simulink model "EV_Modeling"  (R2024b)
settings: Solver=FixedStepAuto  StartTime=0.0  StopTime=3500  FixedStep=0.1  RelTol=1e-3
values from neighbouring files (symbols this model uses):
  battery_SOC_resistance = battery_SOC(:,3)    [EV_Truck.m]
  battery_SOC_SOC = battery_SOC(:,1)    [EV_Truck.m]    (also in simulink.m)
  battery_SOC_voltage = battery_SOC(:,2)    [EV_Truck.m]    (also in simulink.m)
  electric_consumption_ressistancce = electric_consumption(:,2)    [EV_Truck.m]    (also in simulink.m)
  electric_consumption_voltage = electric_consumption(:,1)    [EV_Truck.m]    (also in simulink.m)
  motor_efficiency_efficiency = table2array(motor_efficiency(2:height(motor_efficiency),2:width(motor_efficiency)))    [EV_Truck.m]    (also in simulink.m)
  motor_efficiency_RPM = table2array(motor_efficiency(2:height(motor_efficiency),1))    [EV_Truck.m]    (also in simulink.m)
  motor_efficiency_torque = transpose(motor_efficiency_torque)    [EV_Truck.m]    (also in simulink.m)
  motor_RPM_torque = table2array(motor_torque(1:14,1))    [EV_Truck.m]    (also in simulink.m)
  motor_torque_RPM = table2array(motor_torque(1:14,2))    [EV_Truck.m]    (also in simulink.m)
undefined symbols (not defined in the file or in its folder): battery_builder_rtmsupport, battery_sli_rtmsupport, DiscIntNeverNeededParam, gcbh, recurrentNet
libraries: dlutilitylib x10, dlsequencelib x10, packLibrary_lib x10, simulink x7, dlconvfclib x6, dlactivationlib x5, sharedTrackingLibrary x3, mpcadaslib x2, nesl_utility x2, fl_lib x2, slpidlib x2, simulink_extras x1
(part 6 of 9)

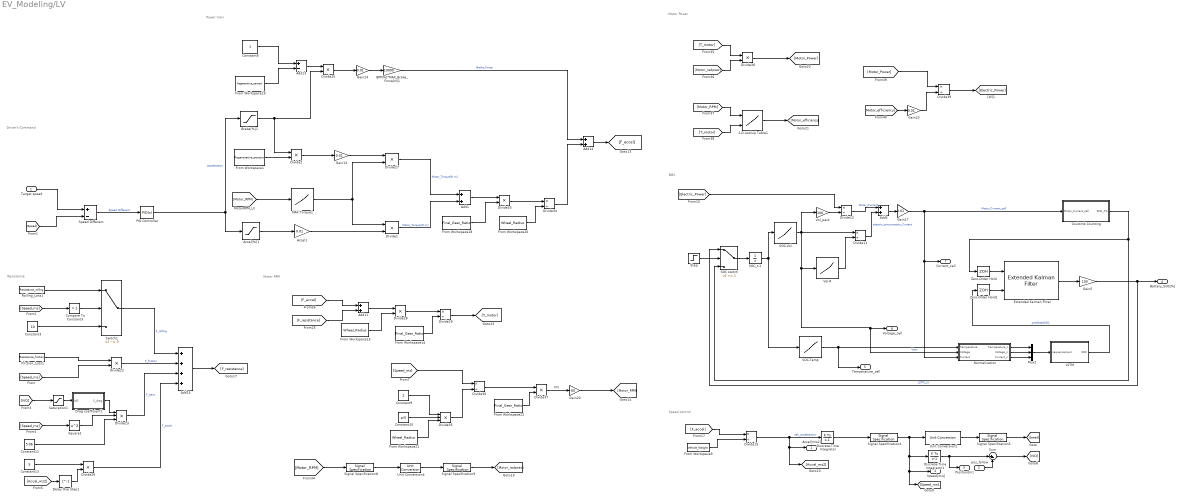
== system EV_Modeling/LV ==
  note: Speed control
  note: Driver's Command
  note: BMS
  note: RPS
  note: Power train
  note: Resistance
  note: Motor RPM
  note: Motor Power
  Target speed : Inport
  pos_follow : Inport  Port=2
  " Normalization" : MATLAB Function  TreatAsAtomicUnit=on
  2-D Lookup Table1 : Lookup_n-D  BreakpointsForDimension1=motor_efficiency_RPM  BreakpointsForDimension2=motor_efficiency_torque  Table=motor_efficiency_efficiency  RemoveProtectionInput=on  InternalRulePriority=Speed  RndMeth=Simplest
      settings: InputPortMap=u0,u1
  Accel1 : Gain  Gain=0.01
  Accel[%]1 : Saturate  UpperLimit=100  LowerLimit=0
  Add{1,4,11,14} (4 alike) : Sum
  Add13 : Sum  Inputs=+-
  Add15 : Sum  Inputs=++++
  BPP[%]*MAX_Brake_Force[N]1 : Gain  Gain=10000
  Brake[%]1 : Saturate  UpperLimit=0  LowerLimit=-100
  Compare To Constant3 : simulink/Logic and Bit Operations/Compare To Constant  relop=>  const=1  OutDataTypeStr=boolean
  Constant10 : Constant  Value=pi()
  Constant12 : Constant  Value=5.06
  Constant13 : Constant  Value=5
  Constant3 : Constant  Value=10
  Constant8 : Constant
  Constant9 : Constant  Value=2
  Coulomb Counting : Subsystem
  Delay One Step1 : Delay  DelayLength=1
  Discrete-Time Integrator : DiscreteIntegrator  SampleTime=-1  ICPrevOutput=DiscIntNeverNeededParam  ICPrevScaledInput=DiscIntNeverNeededParam
  Discrete-Time Integrator1 : DiscreteIntegrator  SampleTime=-1  ICPrevOutput=DiscIntNeverNeededParam  ICPrevScaledInput=DiscIntNeverNeededParam
  Divide{1..2,22,25..28,33,37..38} (10 alike) : Product  Inputs=**
  Divide{11..12,15,29,34,36,39} (7 alike) : Product  Inputs=*/
  Divide23 : Product  Inputs=***
  Divide35 : Product  Inputs=***
  Drag coefficient1 : MATLAB Function  TreatAsAtomicUnit=on
  Extended Kalman Filter : sharedTrackingLibrary/Extended Kalman Filter  StateTransitionFcn=myStateTransitionFcn  HasStateTransitionJacobianFcn=off  HasAdditiveProcessNoise=Additive  ProcessNoise=0.0005  HasTimeVaryingProcessNoise=off  HasStateTransitionFcnExtraArgument=1  InitialState=1  InitialStateCovariance=0.02  MeasurementFcn1=myMeasurementFcn  HasMeasurementJacobianFcn1=off  HasMeasurementEnablePort1=off  HasAdditiveMeasurementNoise1=Additive  MeasurementNoise1=0.01  HasTimeVaryingMeasurementNoise1=off  HasMeasurementFcnExtraArgument1=0  HasMeasurementWrapping1=off  MeasurementFcn2=myMeasurementFcn  HasMeasurementJacobianFcn2=off  HasMeasurementEnablePort2=off  HasAdditiveMeasurementNoise2=Additive  MeasurementNoise2=1  HasTimeVaryingMeasurementNoise2=off  HasMeasurementFcnExtraArgument2=0  HasMeasurementWrapping2=off  MeasurementFcn3=myMeasurementFcn  HasMeasurementJacobianFcn3=off  HasMeasurementEnablePort3=off  HasAdditiveMeasurementNoise3=Additive  MeasurementNoise3=1  HasTimeVaryingMeasurementNoise3=off  HasMeasurementFcnExtraArgument3=0  HasMeasurementWrapping3=off  MeasurementFcn4=myMeasurementFcn  HasMeasurementJacobianFcn4=off  HasMeasurementEnablePort4=off  HasAdditiveMeasurementNoise4=Additive  MeasurementNoise4=1  HasTimeVaryingMeasurementNoise4=off  HasMeasurementFcnExtraArgument4=0  HasMeasurementWrapping4=off  MeasurementFcn5=myMeasurementFcn  HasMeasurementJacobianFcn5=off  HasMeasurementEnablePort5=off  HasAdditiveMeasurementNoise5=Additive  MeasurementNoise5=1  HasTimeVaryingMeasurementNoise5=off  HasMeasurementFcnExtraArgument5=0  HasMeasurementWrapping5=off  EnableMultirate=off  StateTransitionFcnSampleTime=1  MeasurementFcn1SampleTime=1  MeasurementFcn2SampleTime=1  MeasurementFcn3SampleTime=1  MeasurementFcn4SampleTime=1  MeasurementFcn5SampleTime=1  UseCurrentEstimator=on  OutputStateCovariance=off  DataType=double  SampleTime=0.1  NumberOfMeasurements=1
  Friction_Loss1 : FromWorkspace  VariableName=Resistance_friction
  From Workspace1 : FromWorkspace  VariableName=Regenerative_percent
  From Workspace14 : FromWorkspace  VariableName=Final_Gear_Ratio
  From Workspace15 : FromWorkspace  VariableName=Wheel_Radius
  From Workspace18 : FromWorkspace  VariableName=Final_Gear_Ratio
  From Workspace19 : FromWorkspace  VariableName=Regenerative_percent
  From Workspace20 : FromWorkspace  VariableName=Wheel_Radius
  From Workspace21 : FromWorkspace  VariableName=Wheel_Radius
  From Workspace22 : FromWorkspace  VariableName=Final_Gear_Ratio
  From Workspace9 : FromWorkspace  VariableName=Vehicle_Weight
  Gain{13..14,17,23} (4 alike) : Gain  Gain=0.01
  Gain20 : Gain  Gain=60
  Gain5 : Gain  Gain=100
  LSTM : Subsystem  TreatAsAtomicUnit=on
  MAX Torque1 : Lookup_n-D  NumberOfTableDimensions=1  BreakpointsForDimension1=motor_RPM_torque  Table=motor_torque_RPM  RemoveProtectionInput=on  InternalRulePriority=Speed  RndMeth=Simplest
  Mux2 : Mux  Inputs=3
  PID Controller : slpidlib/PID Controller  Controller=PID  Form=Parallel  TimeDomain=Continuous-time  UseExternalTs=off  SampleTime=-1  IntegratorMethod=Forward Euler  FilterMethod=Forward Euler  ControllerParametersSource=internal  P=100  I=0.01  UseKiTs=off  D=0.0001  UseExternalDerivativeSource=off  N=10  UseFilter=on  TunerSelectOption=Transfer Function Based (PID Tuner App)  InitialConditionSource=internal  InitialConditionForIntegrator=0  InitialConditionForFilter=0  DifferentiatorICPrevScaledInput=0  ExternalReset=none  TrackingMode=off  Kt=1  LimitOutput=off  SatLimitsSource=internal  UpperSaturationLimit=inf  LowerSaturationLimit=-inf  LinearizeAsGain=on  AntiWindupMode=none  Kb=1  LimitIntegrator=off  UpperIntegratorSaturationLimit=inf  LowerIntegratorSaturationLimit=-inf  POutMin=[]  POutMax=[]  IOutMin=[]  IOutMax=[]  DOutMin=[]  DOutMax=[]  NOutMin=[]  NOutMax=[]  SumOutMin=[]  SumOutMax=[]  SaturationOutMin=[]  SaturationOutMax=[]  PParamMin=[]  PParamMax=[]  IParamMin=[]  IParamMax=[]  DParamMin=[]  DParamMax=[]  NParamMin=[]  NParamMax=[]  KbParamMin=[]  KbParamMax=[]  KtParamMin=[]  KtParamMax=[]  KbOutMin=[]  KbOutMax=[]  KtOutMin=[]  KtOutMax=[]  IntegratorOutMin=[]  IntegratorOutMax=[]  FilterOutMin=[]  FilterOutMax=[]  SumI1OutMin=[]  SumI1OutMax=[]  SumI2OutMin=[]  SumI2OutMax=[]  SumI3OutMin=[]  SumI3OutMax=[]  SumI4OutMin=[]  SumI4OutMax=[]  SumDOutMin=[]  SumDOutMax=[]  DifferentiatorOutMin=[]  DifferentiatorOutMax=[]  FilterDiffOutCoefMin=[]  FilterDiffOutCoefMax=[]  ReciprocalOutMin=[]  ReciprocalOutMax=[]  SumDenOutMin=[]  SumDenOutMax=[]  SumNumOutMin=[]  SumNumOutMax=[]  DivideOutMin=[]  DivideOutMax=[]  UdiffTsProdOutMin=[]  UdiffTsProdOutMax=[]  NTsProdOutMin=[]  NTsProdOutMax=[]  UintegralTsProdOutMin=[]  UintegralTsProdOutMax=[]  UngainTsProdOutMin=[]  UngainTsProdOutMax=[]  ClampingZeroOutDataTypeStr=Inherit: Inherit via back propagation  ClampingZeroOutMin=[]  ClampingZeroOutMax=[]  FilterDenConstantOutDataTypeStr=Inherit: Inherit via back propagation  FilterDenConstantOutMin=[]  FilterDenConstantOutMax=[]  PCopyOutDataTypeStr=Inherit: Inherit via back propagation  PCopyOutMin=[]  PCopyOutMax=[]  NCopyOutDataTypeStr=Inherit: Inherit via back propagation  NCopyOutMin=[]  NCopyOutMax=[]  IntegratorContinuousStateAttributes=''  IntegratorStateMustResolveToSignalObject=off  IntegratorRTWStateStorageClass=Auto  FilterContinuousStateAttributes=''  FilterStateMustResolveToSignalObject=off  FilterRTWStateStorageClass=Auto  ParallelPVariant=InternalParameters  IdealPVariant=Disabled  IVariant=InternalParameters  DVariant=InternalParameters  IntegratorVariant=Continuous  SatVariant=Disabled  AWVariant=Passthrough  PCopyVariant=Disabled  TRVariant=Disabled  FdbkBlocksVariant=Forward  IdealPFdbkVariant=Disabled  SatFdbkVariant=Disabled  DerivativeFilterVariant=ContFilter  NVariant=InternalParameters  NCopyVariant=Disabled  FilterICVariant=InternalICsFilter  IntegratorICVariant=InternalICs  ExternalResetVariant=Disabled  TRSumVariant=Passthrough  SumFdbkVariant=Disabled  SumVariant=Sum_PID  TsampFilterVariant=InternalTs  TsampNgainVariant=Passthrough  TsampIntegralVariant=Disabled_SignalSpec  ExternalSaturationOutDataTypeStr=Inherit: Same as second input  DerivativeSourceVariant=ErrorSignal  PreIntVariant=InternalPreInt
  Rolling_Loss1 : FromWorkspace  VariableName=Resistance_rolling
  SOC switch : Switch  Threshold=1  SaturateOnIntegerOverflow=off  InputSameDT=off
  SOC-Temp : Lookup_n-D  NumberOfTableDimensions=1  BreakpointsForDimension1=|  Table=|  RemoveProtectionInput=on  InternalRulePriority=Speed  RndMeth=Simplest
      BreakpointsForDimension1=|
      | [6.4447
      | 6.4638
      | 6.4868
      | 6.5167
      | 6.5496
      | 6.5844
      | 6.6191
      | 6.6540
      | 6.6892
      | 6.7216
      | 6.7487
      | 6.7726
      | 6.7942
      | 6.8095
      | 6.8230
      | 6.8389
      | 6.8609
      | 6.8840
      | 6.9099
      | 6.9359
      | 6.9619
      | 6.9880
      | 7.0141
      | 7.0403
      | 7.0668
      | 7.0938
      | 7.1216
      | 7.1470
      | 7.1716
      | 7.1939
      | 7.2180
      | 7.2387
      | 7.2584
      | 7.2753
      | 7.2920
      | 7.3083
      | 7.3306
      | 7.3535
      | 7.3781
      | 7.4059
      | 7.4419
      | 7.4845
      | 7.5268
      | 7.5689
      | 7.6108
      | 7.6525
      | 7.6940
      | 7.7352
      | 7.7763
      | 7.8171
      | 7.8578
      | 7.8982
      | 7.9384
      | 7.9784
      | 8.0181
      | 8.0577
      | 8.0970
      | 8.1362
      | 8.1751
      | 8.2138
      | 8.2523
      | 8.2905
      | 8.3285
      | 8.3664
      | 8.4039
      | 8.4413
      | 8.4785
      | 8.5155
      | 8.5523
      | 8.5890
      | 8.6254
      | 8.6616
      | 8.6976
      | 8.7334
      | 8.7689
      | 8.8043
      | 8.8396
      | 8.8747
      | 8.9096
      | 8.9444
      | 8.9790
      | 9.0135
      | 9.0478
      | 9.0819
      | 9.1159
      | 9.1498
      | 9.1835
      | 9.2170
      | 9.2504
      | 9.2837
      | 9.3168
      | 9.3497
      | 9.3825
      | 9.3960
      | 9.3992
      | 9.4037
      | 9.4061
      | 9.4082
      | 9.4128
      | 9.4152
      | 9.4175
      | 9.4180
      | 9.4222
      | 9.4269
      | 9.4284
      | 9.4316
      | 9.4363
      | 9.4411
      | 9.4412
      | 9.4458
      | 9.4476
      | 9.4505
      | 9.4541
      | 9.4552
      | 9.4598
      | 9.4644
      | 9.4669
      | 9.4689
      | 9.4733
      | 9.4795
      | 9.4914
      | 9.5010
      | 9.5039
      | 9.5086
      | 9.5183
      | 9.5279
      | 9.5303
      | 9.5331
      | 9.5514
      | 9.5708
      | 9.5931
      | 9.6158
      | 9.6397
      | 9.6657
      | 9.6961
      | 9.7278
      | 9.7583
      | 9.7778
      | 9.8006
      | 9.8249
      | 9.8483
      | 9.8700
      | 9.8920
      | 9.9150
      | 9.9398
      | 9.9684
      | 10.0008
      | 10.0298
      | 10.0557
      | 10.0789
      | 10.1006
      | 10.1179
      | 10.1358
      | 10.1555
      | 10.1729
      | 10.1913
      | 10.2119
      | 10.2322
      | 10.2514
      | 10.2738
      | 10.2977
      | 10.3288
      | 10.3629
      | 10.3997
      | 10.4363
      | 10.4692
      | 10.5009
      | 10.5342
      | 10.5672
      | 10.6002
      | 10.6333
      | 10.6631
      | 10.6973
      | 10.7324
      | 10.7675
      | 10.8023
      | 10.8340
      | 10.8391
      | 10.8430
      | 10.8474
      | 10.8505
      | 10.8518
      | 10.8535
      | 10.8563
      | 10.8774
      | 10.9089
      | 10.9346
      | 10.9554
      | 10.9735
      | 10.9893
      | 11.0052
      | 11.0213
      | 11.0308
      | 11.0340
      | 11.0394
      | 11.0512
      | 11.0741
      | 11.1046
      | 11.1356
      | 11.1677
      | 11.1989
      | 11.2237
      | 11.2423
      | 11.2528
      | 11.2660
      | 11.2871
      | 11.3222
      | 11.3576
      | 11.3928
      | 11.4037
      | 11.4077
      | 11.4119
      | 11.4153
      | 11.4161
      | 11.4181
      | 11.4204
      | 11.4313
      | 11.4465
      | 11.4588
      | 11.4698
      | 11.4768
      | 11.4788
      | 11.4805
      | 11.4885
      | 11.5071
      | 11.5280
      | 11.5527
      | 11.5813
      | 11.6135
      | 11.6461
      | 11.6717
      | 11.6986
      | 11.7283
      | 11.7633
      | 11.7957
      | 11.8258
      | 11.8591
      | 11.8879
      | 11.9147
      | 11.9416
      | 11.9725
      | 12.0081
      | 12.0436
      | 12.0789
      | 12.1141
      | 12.1491
      | 12.1708
      | 12.1744
      | 12.1765
      | 12.1781
      | 12.1818
      | 12.1840
      | 12.1857
      | 12.1898
      | 12.1938
      | 12.1955
      | 12.1980
      | 12.2023
      | 12.2066
      | 12.2109
      | 12.2173
      | 12.2395
      | 12.2628
      | 12.2840
      | 12.3054
      | 12.3268
      | 12.3524
      | 12.3787
      | 12.4065
      | 12.4295
      | 12.4440
      | 12.4532
      | 12.4611
      | 12.4721
      | 12.4852
      | 12.4966
      | 12.5105
      | 12.5242
      | 12.5440
      | 12.5669
      | 12.5906
      | 12.6162
      | 12.6416
      | 12.6665
      | 12.6906
      | 12.7130
      | 12.7222
      | 12.7245
      | 12.7270
      | 12.7297
      | 12.7300
      | 12.7325
      | 12.7354
      | 12.7384
      | 12.7623
      | 12.8010
      | 12.8391
      | 12.8764
      | 12.9088
      | 12.9386
      | 12.9709
      | 13.0077
      | 13.0465
      | 13.0837
      | 13.1173
      | 13.1471
      | 13.1767
      | 13.2022
      | 13.2226
      | 13.2403
      | 13.2572
      | 13.2719
      | 13.2801
      | 13.2843
      | 13.2867
      | 13.2959
      | 13.3092
      | 13.3263
      | 13.3526
      | 13.3813
      | 13.4073
      | 13.4319
      | 13.4524
      | 13.4680
      | 13.4914
      | 13.5186
      | 13.5530
      | 13.5867
      | 13.6189
      | 13.6522
      | 13.6841
      | 13.7134
      | 13.7373
      | 13.7571
      | 13.7720
      | 13.7797
      | 13.7964
      | 13.8300
      | 13.8690
      | 13.9077
      | 13.9462
      | 13.9846
      | 14.0227
      | 14.0606
      | 14.0982
      | 14.1353
      | 14.1537
      | 14.1558
      | 14.1581
      | 14.1583
      | 14.1605
      | 14.1631
      | 14.1658
      | 14.1667
      | 14.1686
      | 14.1716
      | 14.1746
      | 14.1778
      | 14.1898
      | 14.2301
      | 14.2701
      | 14.3099
      | 14.3495
      | 14.3889
      | 14.4281
      | 14.4671
      | 14.5059
      | 14.5444
      | 14.5828
      | 14.6209
      | 14.6588
      | 14.6965
      | 14.7340
      | 14.7712
      | 14.8083
      | 14.8452
      | 14.8788
      | 14.8994
      | 14.9073
      | 14.9080
      | 14.9111
      | 14.9134
      | 14.9144
      | 14.9284
      | 14.9534
      | 14.9854
      | 15.0229
      | 15.0531
      | 15.0770
      | 15.0942
      | 15.1109
      | 15.1260
      | 15.1365
      | 15.1478
      | 15.1612
      | 15.1804
      | 15.2019
      | 15.2229
      | 15.2476
      | 15.2752
      | 15.3049
      | 15.3387
      | 15.3665
      | 15.3893
      | 15.4086
      | 15.4243
      | 15.4365
      | 15.4383
      | 15.4387
      | 15.4420
      | 15.4464
      | 15.4539
      | 15.4627
      | 15.4749
      | 15.4897
      | 15.5042
      | 15.5246
      | 15.5473
      | 15.5692
      | 15.5944
      | 15.6174
      | 15.6401
      | 15.6617
      | 15.6803
      | 15.6980
      | 15.7129
      | 15.7274
      | 15.7403
      | 15.7559
      | 15.7717
      | 15.7879
      | 15.7978
      | 15.8120
      | 15.8306
      | 15.8465
      | 15.8622
      | 15.8773
      | 15.8976
      | 15.9176
      | 15.9368
      | 15.9535
      | 15.9709
      | 15.9896
      | 16.0121
      | 16.0371
      | 16.0614
      | 16.0841
      | 16.1095
      | 16.1350
      | 16.1604
      | 16.1858
      | 16.2113
      | 16.2367
      | 16.2622
      | 16.2877
      | 16.3133
      | 16.3391
      | 16.3651
      | 16.3917
      | 16.4194
      | 16.4489
      | 16.4784
      | 16.5078
      | 16.5371
      | 16.5663
      | 16.5953
      | 16.6241
      | 16.6523
      | 16.6797
      | 16.7091
      | 16.7389
      | 16.7693
      | 16.8010
      | 16.8352
      | 16.8671
      | 16.8945
      | 16.9208
      | 16.9451
      | 16.9694
      | 16.9938
      | 17.0180
      | 17.0422
      | 17.0661
      | 17.0894
      | 17.1109
      | 17.1348
      | 17.1578
      | 17.1783
      | 17.1994
      | 17.2219
      | 17.2413
      | 17.2590
      | 17.2796
      | 17.3005
      | 17.3221
      | 17.3457
      | 17.3671
      | 17.3900
      | 17.4160
      | 17.4429
      | 17.4678
      | 17.4929
      | 17.5180
      | 17.5434
      | 17.5693
      | 17.5962
      | 17.6209
      | 17.6457
      | 17.6703
      | 17.6944
      | 17.7176
      | 17.7377
      | 17.7573
      | 17.7750
      | 17.7878
      | 17.8017
      | 17.8180
      | 17.8338
      | 17.8407
      | 17.8525
      | 17.8701
      | 17.8812
      | 17.8967
      | 17.9161
      | 17.9387
      | 17.9618
      | 17.9865
      | 18.0144
      | 18.0431
      | 18.0733
      | 18.1029
      | 18.1311
      | 18.1606
      | 18.1889
      | 18.2144
      | 18.2382
      | 18.2648
      | 18.2914
      | 18.3178
      | 18.3439
      | 18.3692
      | 18.3922
      | 18.4167
      | 18.4443
      | 18.4726
      | 18.5022
      | 18.5305
      | 18.5602
      | 18.5888
      | 18.6153
      | 18.6416
      | 18.6675
      | 18.6924
      | 18.7146
      | 18.7368
      | 18.7592
      | 18.7819
      | 18.8053
      | 18.8305
      | 18.8527
      | 18.8748
      | 18.8962
      | 18.9159
      | 18.9384
      | 18.9606
      | 18.9819
      | 19.0008
      | 19.0208
      | 19.0436
      | 19.0724
      | 19.1056
      | 19.1430
      | 19.1844
      | 19.2234
      | 19.2618
      | 19.3021
      | 19.3368
      | 19.3673
      | 19.3973
      | 19.4266
      | 19.4546
      | 19.4795
      | 19.5018
      | 19.5247
      | 19.5489
      | 19.5760
      | 19.6036
      | 19.6320
      | 19.6619
      | 19.6945
      | 19.7318
      | 19.7708
      | 19.8102
      | 19.8475
      | 19.8806
      | 19.9092
      | 19.9250
      | 19.9389
      | 19.9547
      | 19.9755
      | 19.9950
      | 20.0182
      | 20.0479
      | 20.0806
      | 20.1151
      | 20.1496
      | 20.1842
      | 20.2191
      | 20.2513
      | 20.2783
      | 20.3024
      | 20.3243
      | 20.3401
      | 20.3542
      | 20.3706
      | 20.3928
      | 20.4161
      | 20.4421
      | 20.4682
      | 20.4942
      | 20.5203
      | 20.5465
      | 20.5728
      | 20.5994
      | 20.6264
      | 20.6542
      | 20.6797
      | 20.7044
      | 20.7270
      | 20.7511
      | 20.7722
      | 20.7922
      | 20.8095
      | 20.8267
      | 20.8435
      | 20.8660
      | 20.8891
      | 20.9138
      | 20.9416
      | 20.9772
      | 21.0192
      | 21.0609
      | 21.1024
      | 21.1437
      | 21.1848
      | 21.2258
      | 21.2665
      | 21.3070
      | 21.3473
      | 21.3874
      | 21.4273
      | 21.4670
      | 21.5065
      | 21.5458
      | 21.5849
      | 21.6237
      | 21.6624
      | 21.7009
      | 21.7391
      | 21.7772
      | 21.8150
      | 21.8526
      | 21.8900
      | 21.9272
      | 21.9642
      | 22.0010
      | 22.0376
      | 22.0741
      | 22.1104
      | 22.1464
      | 22.1823
      | 22.2180
      | 22.2534
      | 22.2887
      | 22.3238
      | 22.3587
      | 22.3935
      | 22.4282
      | 22.4627
      | 22.4970
      | 22.5312
      | 22.5653
      | 22.5992
      | 22.6330
      | 22.6666
      | 22.7000
      | 22.7334
      | 22.7666
      | 22.7996
      | 22.8325
      | 22.8652
      | 22.8978
      | 22.9303
      | 22.9337
      | 22.9348
      | 22.9356
      | 22.9387
      | 22.9419
      | 22.9452
      | 22.9456
      | 22.9485
      | 22.9519
      | 22.9553
      | 22.9582
      | 22.9587
      | 22.9621
      | 22.9626
      | 22.9655
      | 22.9688
      | 22.9693
      | 22.9722
      | 22.9756
      | 22.9788
      | 22.9821
      | 22.9828
      | 22.9853
      | 22.9884
      | 22.9963
      | 23.0097
      | 23.0230
      | 23.0355
      | 23.0459
      | 23.0498
      | 23.0555
      | 23.0659
      | 23.0762
      | 23.0797
      | 23.0835
      | 23.1022
      | 23.1220
      | 23.1445
      | 23.1674
      | 23.1914
      | 23.2176
      | 23.2479
      | 23.2794
      | 23.3098
      | 23.3297
      | 23.3527
      | 23.3771
      | 23.4008
      | 23.4226
      | 23.4450
      | 23.4681
      | 23.4931
      | 23.5216
      | 23.5539
      | 23.5829
      | 23.6088
      | 23.6322
      | 23.6542
      | 23.6719
      | 23.6902
      | 23.7102
      | 23.7282
      | 23.7469
      | 23.7679
      | 23.7885
      | 23.8080
      | 23.8306
      | 23.8547
      | 23.8857
      | 23.9196
      | 23.9560
      | 23.9922
      | 24.0249
      | 24.0565
      | 24.0895
      | 24.1224
      | 24.1552
      | 24.1881
      | 24.2178
      | 24.2517
      | 24.2866
      | 24.3214
      | 24.3559
      | 24.3875
      | 24.3993
      | 24.4019
      | 24.4049
      | 24.4074
      | 24.4080
      | 24.4112
      | 24.4114
      | 24.4383
      | 24.4697
      | 24.4955
      | 24.5166
      | 24.5351
      | 24.5514
      | 24.5678
      | 24.5844
      | 24.5946
      | 24.5989
      | 24.6052
      | 24.6177
      | 24.6408
      | 24.6712
      | 24.7021
      | 24.7340
      | 24.7651
      | 24.7901
      | 24.8091
      | 24.8202
      | 24.8341
      | 24.8555
      | 24.8903
      | 24.9254
      | 24.9603
      | 24.9777
      | 24.9804
      | 24.9832
      | 24.9857
      | 24.9861
      | 24.9891
      | 24.9899
      | 25.0065
      | 25.0222
      | 25.0352
      | 25.0468
      | 25.0547
      | 25.0578
      | 25.0606
      | 25.0694
      | 25.0884
      | 25.1095
      | 25.1345
      | 25.1630
      | 25.1951
      | 25.2274
      | 25.2532
      | 25.2802
      | 25.3097
      | 25.3445
      | 25.3767
      | 25.4068
      | 25.4398
      | 25.4686
      | 25.4955
      | 25.5224
      | 25.5532
      | 25.5885
      | 25.6237
      | 25.6588
      | 25.6937
      | 25.7284
      | 25.7630
      | 25.7631
      | 25.7653
      | 25.7677
      | 25.7697
      | 25.7702
      | 25.7728
      | 25.7755
      | 25.7783
      | 25.7811
      | 25.7840
      | 25.7870
      | 25.7891
      | 25.7900
      | 25.8111
      | 25.8336
      | 25.8571
      | 25.8786
      | 25.9002
      | 25.9219
      | 25.9477
      | 25.9741
      | 26.0019
      | 26.0251
      | 26.0402
      | 26.0501
      | 26.0589
      | 26.0706
      | 26.0843
      | 26.0963
      | 26.1109
      | 26.1251
      | 26.1454
      | 26.1684
      | 26.1924
      | 26.2181
      | 26.2435
      | 26.2686
      | 26.2929
      | 26.3155
      | 26.3330
      | 26.3336
      | 26.3346
      | 26.3359
      | 26.3373
      | 26.3388
      | 26.3405
      | 26.3422
      | 26.3732
      | 26.4115
      | 26.4492
      | 26.4861
      | 26.5184
      | 26.5481
      | 26.5802
      | 26.6167
      | 26.6551
      | 26.6919
      | 26.7253
      | 26.7550
      | 26.7846
      | 26.8102
      | 26.8310
      | 26.8491
      | 26.8664
      | 26.8817
      | 26.8908
      | 26.8960
      | 26.8971
      | 26.9006
      | 26.9105
      | 26.9244
      | 26.9420
      | 26.9684
      | 26.9971
      | 27.0232
      | 27.0479
      | 27.0688
      | 27.0848
      | 27.1084
      | 27.1358
      | 27.1699
      | 27.2034
      | 27.2355
      | 27.2686
      | 27.3003
      | 27.3296
      | 27.3536
      | 27.3738
      | 27.3892
      | 27.3979
      | 27.4150
      | 27.4484
      | 27.4869
      | 27.5252
      | 27.5634
      | 27.6013
      | 27.6390
      | 27.6765
      | 27.7138
      | 27.7505
      | 27.7810
      | 27.7818
      | 27.7829
      | 27.7840
      | 27.7853
      | 27.7865
      | 27.7868
      | 27.7883
      | 27.7900
      | 27.7918
      | 27.7936
      | 27.8179
      | 27.8577
      | 27.8972
      | 27.9366
      | 27.9758
      | 28.0147
      | 28.0535
      | 28.0920
      | 28.1304
      | 28.1685
      | 28.2065
      | 28.2442
      | 28.2818
      | 28.3191
      | 28.3562
      | 28.3931
      | 28.4299
      | 28.4664
      | 28.4998
      | 28.5208
      | 28.5337
      | 28.5341
      | 28.5353
      | 28.5355
      | 28.5375
      | 28.5556
      | 28.5807
      | 28.6125
      | 28.6497
      | 28.6798
      | 28.7039
      | 28.7216
      | 28.7387
      | 28.7544
      | 28.7657
      | 28.7777
      | 28.7917
      | 28.8113
      | 28.8331
      | 28.8544
      | 28.8792
      | 28.9068
      | 28.9365
      | 28.9701
      | 28.9980
      | 29.0210
      | 29.0407
      | 29.0569
      | 29.0697
      | 29.0726
      | 29.0742
      | 29.0785
      | 29.0839
      | 29.0923
      | 29.1018
      | 29.1148
      | 29.1301
      | 29.1451
      | 29.1659
      | 29.1889
      | 29.2110
      | 29.2363
      | 29.2596
      | 29.2825
      | 29.3044
      | 29.3234
      | 29.3416
      | 29.3571
      | 29.3721
      | 29.3857
      | 29.4018
      | 29.4181
      | 29.4348
      | 29.4454
      | 29.4603
      | 29.4793
      | 29.4957
      | 29.5119
      | 29.5276
      | 29.5482
      | 29.5686
      | 29.5882
      | 29.6054
      | 29.6232
      | 29.6423
      | 29.6650
      | 29.6902
      | 29.7147
      | 29.7377
      | 29.7632
      | 29.7888
      | 29.8144
      | 29.8399
      | 29.8655
      | 29.8911
      | 29.9167
      | 29.9423
      | 29.9681
      | 29.9940
      | 30.0201
      | 30.0468
      | 30.0745
      | 30.1040
      | 30.1335
      | 30.1629
      | 30.1922
      | 30.2213
      | 30.2503
      | 30.2791
      | 30.3073
      | 30.3347
      | 30.3642
      | 30.3939
      | 30.4243
      | 30.4559
      | 30.4898
      | 30.5216
      | 30.5490
      | 30.5755
      | 30.6000
      | 30.6245
      | 30.6490
      | 30.6734
      | 30.6978
      | 30.7219
      | 30.7455
      | 30.7672
      | 30.7913
      | 30.8145
      | 30.8354
      | 30.8568
      | 30.8796
      | 30.8993
      | 30.9175
      | 30.9384
      | 30.9597
      | 30.9816
      | 31.0054
      | 31.0271
      | 31.0502
      | 31.0763
      | 31.1033
      | 31.1284
      | 31.1536
      | 31.1789
      | 31.2044
      | 31.2305
      | 31.2574
      | 31.2823
      | 31.3072
      | 31.3320
      | 31.3564
      | 31.3797
      | 31.4002
      | 31.4202
      | 31.4383
      | 31.4518
      | 31.4663
      | 31.4831
      | 31.4995
      | 31.5072
      | 31.5197
      | 31.5378
      | 31.5496
      | 31.5656
      | 31.5855
      | 31.6083
      | 31.6317
      | 31.6565
      | 31.6844
      | 31.7131
      | 31.7433
      | 31.7729
      | 31.8011
      | 31.8306
      | 31.8589
      | 31.8846
      | 31.9086
      | 31.9353
      | 31.9619
      | 31.9885
      | 32.0147
      | 32.0401
      | 32.0634
      | 32.0881
      | 32.1157
      | 32.1441
      | 32.1736
      | 32.2020
      | 32.2316
      | 32.2602
      | 32.2868
      | 32.3132
      | 32.3393
      | 32.3644
      | 32.3868
      | 32.4093
      | 32.4320
      | 32.4550
      | 32.4786
      | 32.5039
      | 32.5264
      | 32.5487
      | 32.5705
      | 32.5905
      | 32.6133
      | 32.6357
      | 32.6574
      | 32.6767
      | 32.6971
      | 32.7201
      | 32.7489
      | 32.7820
      | 32.8191
      | 32.8599
      | 32.8986
      | 32.9366
      | 32.9765
      | 33.0109
      | 33.0413
      | 33.0713
      | 33.1006
      | 33.1286
      | 33.1537
      | 33.1763
      | 33.1995
      | 33.2238
      | 33.2511
      | 33.2787
      | 33.3072
      | 33.3370
      | 33.3694
      | 33.4064
      | 33.4450
      | 33.4841
      | 33.5210
      | 33.5539
      | 33.5825
      | 33.5989
      | 33.6134
      | 33.6298
      | 33.6509
      | 33.6708
      | 33.6942
      | 33.7239
      | 33.7565
      | 33.7907
      | 33.8250
      | 33.8594
      | 33.8941
      | 33.9262
      | 33.9533
      | 33.9776
      | 33.9997
      | 34.0161
      | 34.0308
      | 34.0477
      | 34.0702
      | 34.0937
      | 34.1199
      | 34.1461
      | 34.1723
      | 34.1985
      | 34.2248
      | 34.2512
      | 34.2779
      | 34.3050
      | 34.3329
      | 34.3585
      | 34.3834
      | 34.4062
      | 34.4306
      | 34.4520
      | 34.4724
      | 34.4902
      | 34.5079
      | 34.5251
      | 34.5479
      | 34.5713
      | 34.5961
      | 34.6239
      | 34.6593
      | 34.7007
      | 34.7420
      | 34.7830
      | 34.8238
      | 34.8645
      | 34.9049
      | 34.9452
      | 34.9853
      | 35.0251
      | 35.0648
      | 35.1043
      | 35.1436
      | 35.1827
      | 35.2216
      | 35.2603
      | 35.2988
      | 35.3371
      | 35.3752
      | 35.4131
      | 35.4508
      | 35.4883
      | 35.5256
      | 35.5627
      | 35.5996
      | 35.6363
      | 35.6728
      | 35.7091
      | 35.7453
      | 35.7813
      | 35.8171
      | 35.8527
      | 35.8881
      | 35.9234
      | 35.9584
      | 35.9933
      | 36.0280
      | 36.0626
      | 36.0971
      | 36.1314
      | 36.1655
      | 36.1996
      | 36.2334
      | 36.2672
      | 36.3008
      | 36.3342
      | 36.3675
      | 36.4007
      | 36.4338
      | 36.4667
      | 36.4994
      | 36.5321
      | 36.5645
      | 36.5969
      | 36.6225
      | 36.6231
      | 36.6247
      | 36.6250
      | 36.6269
      | 36.6289
      | 36.6291
      | 36.6309
      | 36.6329
      | 36.6350
      | 36.6363
      | 36.6371
      | 36.6391
      | 36.6412
      | 36.6433
      | 36.6454
      | 36.6474
      | 36.6494
      | 36.6495
      | 36.6513
      | 36.6532
      | 36.6550
      | 36.6614
      | 36.6755
      | 36.6896
      | 36.7037
      | 36.7176
      | 36.7308
      | 36.7420
      | 36.7469
      | 36.7535
      | 36.7647
      | 36.7758
      | 36.7803
      | 36.7852
      | 36.8043
      | 36.8245
      | 36.8472
      | 36.8705
      | 36.8947
      | 36.9209
      | 36.9512
      | 36.9827
      | 37.0130
      | 37.0333
      | 37.0566
      | 37.0812
      | 37.1051
      | 37.1273
      | 37.1499
      | 37.1733
      | 37.1984
      | 37.2271
      | 37.2592
      | 37.2882
      | 37.3143
      | 37.3380
      | 37.3602
      | 37.3784
      | 37.3972
      | 37.4176
      | 37.4360
      | 37.4551
      | 37.4765
      | 37.4974
      | 37.5174
      | 37.5402
      | 37.5645
      | 37.5955
      | 37.6292
      | 37.6654
      | 37.7013
      | 37.7339
      | 37.7654
      | 37.7983
      | 37.8311
      | 37.8637
      | 37.8965
      | 37.9263
      | 37.9600
      | 37.9947
      | 38.0292
      | 38.0636
      | 38.0950
      | 38.1135
      | 38.1148
      | 38.1154
      | 38.1165
      | 38.1183
      | 38.1202
      | 38.1263
      | 38.1533
      | 38.1846
      | 38.2106
      | 38.2320
      | 38.2510
      | 38.2679
      | 38.2848
      | 38.3019
      | 38.3129
      | 38.3181
      | 38.3254
      | 38.3386
      | 38.3619
      | 38.3923
      | 38.4231
      | 38.4550
      | 38.4860
      | 38.5112
      | 38.5306
      | 38.5425
      | 38.5570
      | 38.5788
      | 38.6134
      | 38.6482
      | 38.6829
      | 38.7067
      | 38.7082
      | 38.7085
      | 38.7097
      | 38.7113
      | 38.7130
      | 38.7197
      | 38.7368
      | 38.7530
      | 38.7667
      | 38.7791
      | 38.7878
      | 38.7920
      | 38.7958
      | 38.8055
      | 38.8249
      | 38.8464
      | 38.8715
      | 38.9001
      | 38.9321
      | 38.9643
      | 38.9903
      | 39.0173
      | 39.0469
      | 39.0815
      | 39.1136
      | 39.1437
      | 39.1766
      | 39.2054
      | 39.2325
      | 39.2594
      | 39.2902
      | 39.3253
      | 39.3603
      | 39.3952
      | 39.4298
      | 39.4644
      | 39.4988
      | 39.5119
      | 39.5129
      | 39.5140
      | 39.5152
      | 39.5165
      | 39.5179
      | 39.5194
      | 39.5195
      | 39.5209
      | 39.5226
      | 39.5242
      | 39.5260
      | 39.5393
      | 39.5616
      | 39.5844
      | 39.6081
      | 39.6300
      | 39.6519
      | 39.6739
      | 39.6998
      | 39.7264
      | 39.7543
      | 39.7778
      | 39.7934
      | 39.8042
      | 39.8137
      | 39.8262
      | 39.8405
      | 39.8533
      | 39.8684
      | 39.8833
      | 39.9039
      | 39.9273
      | 39.9514
      | 39.9773
      | 40.0030
      | 40.0282
      | 40.0527
      | 40.0756
      | 40.0936
      | 40.1023
      | 40.1025
      | 40.1028
      | 40.1032
      | 40.1037
      | 40.1417
      | 40.1797
      | 40.2171
      | 40.2537
      | 40.2859
      | 40.3156
      | 40.3477
      | 40.3839
      | 40.4220
      | 40.4585
      | 40.4918
      | 40.5215
      | 40.5511
      | 40.5769
      | 40.5980
      | 40.6166
      | 40.6344
      | 40.6503
      | 40.6602
      | 40.6664
      | 40.6686
      | 40.6732
      | 40.6839
      | 40.6985
      | 40.7165
      | 40.7430
      | 40.7718
      | 40.7981
      | 40.8230
      | 40.8442
      | 40.8608
      | 40.8847
      | 40.9121
      | 40.9461
      | 40.9794
      | 41.0114
      | 41.0444
      | 41.0761
      | 41.1054
      | 41.1297
      | 41.1503
      | 41.1663
      | 41.1757
      | 41.1934
      | 41.2266
      | 41.2648
      | 41.3028
      | 41.3407
      | 41.3783
      | 41.4157
      | 41.4529
      | 41.4899
      | 41.5264
      | 41.5576
      | 41.5681
      | 41.5683
      | 41.5686
      | 41.5687
      | 41.5690
      | 41.5696
      | 41.5701
      | 41.5752
      | 41.6065
      | 41.6459
      | 41.6851
      | 41.7241
      | 41.7629
      | 41.8015
      | 41.8400
      | 41.8782
      | 41.9162
      | 41.9541
      | 41.9917
      | 42.0291
      | 42.0664
      | 42.1034
      | 42.1403
      | 42.1769
      | 42.2134
      | 42.2497
      | 42.2830
      | 42.3044
      | 42.3195
      | 42.3215
      | 42.3221
      | 42.3227
      | 42.3231
      | 42.3449
      | 42.3702
      | 42.4020
      | 42.4389
      | 42.4690
      | 42.4934
      | 42.5115
      | 42.5292
      | 42.5454
      | 42.5575
      | 42.5702
      | 42.5848
      | 42.6048
      | 42.6270
      | 42.6486
      | 42.6737
      | 42.7014
      | 42.7311
      | 42.7646
      | 42.7926
      | 42.8158
      | 42.8360
      | 42.8527
      | 42.8662
      | 42.8702
      | 42.8729
      | 42.8782
      | 42.8846
      | 42.8938
      | 42.9042
      | 42.9178
      | 42.9338
      | 42.9494
      | 42.9706
      | 42.9938
      | 43.0163
      | 43.0418
      | 43.0653
      | 43.0885
      | 43.1108
      | 43.1302
      | 43.1488
      | 43.1650
      | 43.1806
      | 43.1948
      | 43.2115
      | 43.2284
      | 43.2456
      | 43.2570
      | 43.2725
      | 43.2919
      | 43.3088
      | 43.3256
      | 43.3418
      | 43.3629
      | 43.3837
      | 43.4037
      | 43.4214
      | 43.4397
      | 43.4592
      | 43.4823
      | 43.5076
      | 43.5324
      | 43.5556
      | 43.5814
      | 43.6071
      | 43.6329
      | 43.6586
      | 43.6844
      | 43.7102
      | 43.7360
      | 43.7618
      | 43.7877
      | 43.8138
      | 43.8401
      | 43.8669
      | 43.8947
      | 43.9243
      | 43.9538
      | 43.9832
      | 44.0126
      | 44.0418
      | 44.0708
      | 44.0996
      | 44.1280
      | 44.1555
      | 44.1850
      | 44.2148
      | 44.2451
      | 44.2767
      | 44.3105
      | 44.3422
      | 44.3698
      | 44.3964
      | 44.4211
      | 44.4458
      | 44.4706
      | 44.4953
      | 44.5199
      | 44.5443
      | 44.5680
      | 44.5902
      | 44.6145
      | 44.6380
      | 44.6592
      | 44.6810
      | 44.7041
      | 44.7242
      | 44.7429
      | 44.7642
      | 44.7858
      | 44.8081
      | 44.8321
      | 44.8542
      | 44.8776
      | 44.9039
      | 44.9310
      | 44.9563
      | 44.9817
      | 45.0072
      | 45.0330
      | 45.0592
      | 45.0862
      | 45.1114
      | 45.1365
      | 45.1615
      | 45.1861
      | 45.2098
      | 45.2307
      | 45.2510
      | 45.2697
      | 45.2838
      | 45.2989
      | 45.3163
      | 45.3332
      | 45.3418
      | 45.3550
      | 45.3736
      | 45.3861
      | 45.4028
      | 45.4230
      | 45.4461
      | 45.4698
      | 45.4949
      | 45.5229
      | 45.5517
      | 45.5819
      | 45.6115
      | 45.6398
      | 45.6694
      | 45.6977
      | 45.7236
      | 45.7479
      | 45.7747
      | 45.8015
      | 45.8282
      | 45.8546
      | 45.8802
      | 45.9038
      | 45.9287
      | 45.9565
      | 45.9849
      | 46.0145
      | 46.0430
      | 46.0727
      | 46.1013
      | 46.1281
      | 46.1547
      | 46.1809
      | 46.2062
      | 46.2289
      | 46.2518
      | 46.2748
      | 46.2980
      | 46.3219
      | 46.3474
      | 46.3703
      | 46.3929
      | 46.4150
      | 46.4355
      | 46.4586
      | 46.4814
      | 46.5033
      | 46.5231
      | 46.5439
      | 46.5672
      | 46.5961
      | 46.6291
      | 46.6659
      | 46.7064
      | 46.7447
      | 46.7824
      | 46.8220
      | 46.8562
      | 46.8867
      | 46.9167
      | 46.9461
      | 46.9742
      | 46.9995
      | 47.0224
      | 47.0459
      | 47.0705
      | 47.0979
      | 47.1256
      | 47.1542
      | 47.1841
      | 47.2164
      | 47.2531
      | 47.2915
      | 47.3302
      | 47.3669
      | 47.3997
      | 47.4284
      | 47.4453
      | 47.4605
      | 47.4774
      | 47.4989
      | 47.5192
      | 47.5429
      | 47.5727
      | 47.6052
      | 47.6393
      | 47.6735
      | 47.7077
      | 47.7423
      | 47.7743
      | 47.8016
      | 47.8261
      | 47.8486
      | 47.8655
      | 47.8809
      | 47.8983
      | 47.9211
      | 47.9449
      | 47.9713
      | 47.9977
      | 48.0240
      | 48.0505
      | 48.0769
      | 48.1035
      | 48.1304
      | 48.1576
      | 48.1856
      | 48.2114
      | 48.2366
      | 48.2597
      | 48.2843
      | 48.3061
      | 48.3269
      | 48.3452
      | 48.3634
      | 48.3812
      | 48.4043
      | 48.4279
      | 48.4530
      | 48.4809
      | 48.5160
      | 48.5571
      | 48.5979
      | 48.6386
      | 48.6790
      | 48.7193
      | 48.7594
      | 48.7993
      | 48.8390
      | 48.8785
      | 48.9179
      | 48.9571
      | 48.9960
      | 49.0348
      | 49.0734
      | 49.1118
      | 49.1500
      | 49.1880
      | 49.2259
      | 49.2635
      | 49.3010
      | 49.3382
      | 49.3753
      | 49.4121
      | 49.4488
      | 49.4853
      | 49.5216
      | 49.5577
      | 49.5937
      | 49.6295
      | 49.6651
      | 49.7006
      | 49.7359
      | 49.7709
      | 49.8058
      | 49.8406
      | 49.8752
      | 49.9096
      | 49.9439
      | 49.9781
      | 50.0122
      | 50.0461
      | 50.0799
      | 50.1135
      | 50.1470
      | 50.1804
      | 50.2136
      | 50.2467
      | 50.2797
      | 50.3125
      | 50.3452
      | 50.3778
      | 50.4102
      | 50.4425
      | 50.4747
      | 50.4895
      | 50.4901
      | 50.4907
      | 50.4914
      | 50.4921
      | 50.4929
      | 50.4935
      | 50.4937
      | 50.4945
      | 50.4953
      | 50.4961
      | 50.4969
      | 50.4976
      | 50.4984
      | 50.4991
      | 50.4997
      | 50.5003
      | 50.5009
      | 50.5058
      | 50.5198
      | 50.5324
      | 50.5471
      | 50.5619
      | 50.5767
      | 50.5912
      | 50.6051
      | 50.6171
      | 50.6230
      | 50.6306
      | 50.6425
      | 50.6545
      | 50.6600
      | 50.6658
      | 50.6855
      | 50.7061
      | 50.7291
      | 50.7527
      | 50.7772
      | 50.8036
      | 50.8340
      | 50.8654
      | 50.8958
      | 50.9165
      | 50.9401
      | 50.9650
      | 50.9891
      | 51.0117
      | 51.0346
      | 51.0583
      | 51.0837
      | 51.1124
      | 51.1445
      | 51.1736
      | 51.1999
      | 51.2239
      | 51.2465
      | 51.2652
      | 51.2845
      | 51.3053
      | 51.3242
      | 51.3438
      | 51.3655
      | 51.3869
      | 51.4073
      | 51.4305
      | 51.4550
      | 51.4860
      | 51.5196
      | 51.5556
      | 51.5914
      | 51.6239
      | 51.6555
      | 51.6883
      | 51.7210
      | 51.7536
      | 51.7863
      | 51.8161
      | 51.8497
      | 51.8843
      | 51.9187
      | 51.9530
      | 51.9844
      | 52.0052
      | 52.0096
      | 52.0100
      | 52.0105
      | 52.0110
      | 52.0231
      | 52.0503
      | 52.0816
      | 52.1078
      | 52.1296
      | 52.1491
      | 52.1665
      | 52.1840
      | 52.2017
      | 52.2135
      | 52.2197
      | 52.2279
      | 52.2419
      | 52.2655
      | 52.2960
      | 52.3268
      | 52.3587
      | 52.3897
      | 52.4151
      | 52.4350
      | 52.4477
      | 52.4629
      | 52.4850
      | 52.5194
      | 52.5542
      | 52.5887
      | 52.6146
      | 52.6191
      | 52.6192
      | 52.6194
      | 52.6197
      | 52.6201
      | 52.6327
      | 52.6504
      | 52.6672
      | 52.6816
      | 52.6948
      | 52.7044
      | 52.7096
      | 52.7146
      | 52.7251
      | 52.7450
      | 52.7668
      | 52.7922
      | 52.8209
      | 52.8529
      | 52.8851
      | 52.9113
      | 52.9385
      | 52.9682
      | 53.0026
      | 53.0347
      | 53.0648
      | 53.0977
      | 53.1266
      | 53.1538
      | 53.1810
      | 53.2118
      | 53.2468
      | 53.2816
      | 53.3163
      | 53.3509
      | 53.3854
      | 53.4197
      | 53.4453
      | 53.4454
      | 53.4455
      | 53.4456
      | 53.4458
      | 53.4459
      | 53.4462
      | 53.4466
      | 53.4470
      | 53.4543
      | 53.4746
      | 53.4973
      | 53.5204
      | 53.5444
      | 53.5667
      | 53.5890
      | 53.6114
      | 53.6375
      | 53.6643
      | 53.6923
      | 53.7161
      | 53.7324
      | 53.7439
      | 53.7544
      | 53.7676
      | 53.7826
      | 53.7961
      | 53.8119
      | 53.8274
      | 53.8484
      | 53.8721
      | 53.8966
      | 53.9227
      | 53.9486
      | 53.9741
      | 53.9988
      | 54.0221
      | 54.0406
      | 54.0515
      | 54.0523
      | 54.0531
      | 54.0541
      | 54.0551
      | 54.0564
      | 54.0577
      | 54.0967
      | 54.1344
      | 54.1716
      | 54.2080
      | 54.2402
      | 54.2700
      | 54.3020
      | 54.3380
      | 54.3759
      | 54.4122
      | 54.4454
      | 54.4752
      | 54.5049
      | 54.5309
      | 54.5525
      | 54.5715
      | 54.5899
      | 54.6064
      | 54.6171
      | 54.6243
      | 54.6277
      | 54.6333
      | 54.6448
      | 54.6600
      | 54.6787
      | 54.7053
      | 54.7343
      | 54.7607
      | 54.7859
      | 54.8075
      | 54.8247
      | 54.8489
      | 54.8765
      | 54.9104
      | 54.9436
      | 54.9756
      | 55.0086
      | 55.0403
      | 55.0696
      | 55.0942
      | 55.1153
      | 55.1318
      | 55.1422
      | 55.1603
      | 55.1935
      | 55.2315
      | 55.2692
      | 55.3068
      | 55.3442
      | 55.3814
      | 55.4185
      | 55.4553
      | 55.4915
      | 55.5228
      | 55.5361
      | 55.5367
      | 55.5375
      | 55.5383
      | 55.5392
      | 55.5403
      | 55.5414
      | 55.5427
      | 55.5441
      | 55.5457
      | 55.5532
      | 55.5845
      | 55.6236
      | 55.6625
      | 55.7012
      | 55.7398
      | 55.7781
      | 55.8163
      | 55.8543
      | 55.8921
      | 55.9297
      | 55.9671
      | 56.0043
      | 56.0414
      | 56.0782
      | 56.1149
      | 56.1513
      | 56.1876
      | 56.2238
      | 56.2570
      | 56.2788
      | 56.2946
      | 56.2989
      | 56.2995
      | 56.3002
      | 56.3029
      | 56.3251
      | 56.3507
      | 56.3825
      | 56.4192
      | 56.4494
      | 56.4740
      | 56.4927
      | 56.5109
      | 56.5278
      | 56.5405
      | 56.5540
      | 56.5693
      | 56.5898
      | 56.6123
      | 56.6343
      | 56.6596
      | 56.6876
      | 56.7173
      | 56.7508
      | 56.7789
      | 56.8025
      | 56.8231
      | 56.8404
      | 56.8546
      | 56.8597
      | 56.8635
      | 56.8699
      | 56.8772
      | 56.8873
      | 56.8985
      | 56.9128
      | 56.9294
      | 56.9457
      | 56.9672
      | 56.9908
      | 57.0136
      | 57.0394
      | 57.0633
      | 57.0868
      | 57.1094
      | 57.1294
      | 57.1485
      | 57.1652
      | 57.1815
      | 57.1964
      | 57.2137
      | 57.2311
      | 57.2489
      | 57.2611
      | 57.2772
      | 57.2971
      | 57.3146
      | 57.3320
      | 57.3488
      | 57.3703
      | 57.3915
      | 57.4119
      | 57.4302
      | 57.4490
      | 57.4691
      | 57.4925
      | 57.5181
      | 57.5431
      | 57.5667
      | 57.5927
      | 57.6187
      | 57.6447
      | 57.6707
      | 57.6967
      | 57.7227
      | 57.7487
      | 57.7748
      | 57.8009
      | 57.8272
      | 57.8538
      | 57.8808
      | 57.9088
      | 57.9384
      | 57.9680
      | 57.9975
      | 58.0270
      | 58.0563
      | 58.0855
      | 58.1144
      | 58.1429
      | 58.1706
      | 58.2002
      | 58.2301
      | 58.2605
      | 58.2921
      | 58.3258
      | 58.3575
      | 58.3853
      | 58.4121
      | 58.4371
      | 58.4621
      | 58.4871
      | 58.5121
      | 58.5370
      | 58.5617
      | 58.5858
      | 58.6083
      | 58.6329
      | 58.6567
      | 58.6784
      | 58.7005
      | 58.7240
      | 58.7446
      | 58.7638
      | 58.7855
      | 58.8075
      | 58.8302
      | 58.8545
      | 58.8770
      | 58.9007
      | 58.9272
      | 58.9545
      | 58.9801
      | 59.0058
      | 59.0315
      | 59.0575
      | 59.0839
      | 59.1112
      | 59.1366
      | 59.1620
      | 59.1873
      | 59.2122
      | 59.2362
      | 59.2575
      | 59.2783
      | 59.2975
      | 59.3123
      | 59.3280
      | 59.3460
      | 59.3635
      | 59.3730
      | 59.3869
      | 59.4060
      | 59.4193
      | 59.4365
      | 59.4572
      | 59.4807
      | 59.5047
      | 59.5300
      | 59.5582
      | 59.5871
      | 59.6174
      | 59.6471
      | 59.6756
      | 59.7052
      | 59.7338
      | 59.7599
      | 59.7845
      | 59.8115
      | 59.8385
      | 59.8654
      | 59.8920
      | 59.9179
      | 59.9418
      | 59.9670
      | 59.9950
      | 60.0235
      | 60.0532
      | 60.0818
      | 60.1116
      | 60.1404
      | 60.1674
      | 60.1942
      | 60.2206
      | 60.2462
      | 60.2693
      | 60.2925
      | 60.3159
      | 60.3395
      | 60.3637
      | 60.3894
      | 60.4126
      | 60.4357
      | 60.4581
      | 60.4791
      | 60.5025
      | 60.5256
      | 60.5480
      | 60.5682
      | 60.5895
      | 60.6131
      | 60.6421
      | 60.6751
      | 60.7118
      | 60.7519
      | 60.7901
      | 60.8276
      | 60.8668
      | 60.9010
      | 60.9315
      | 60.9617
      | 60.9912
      | 61.0194
      | 61.0450
      | 61.0683
      | 61.0921
      | 61.1170
      | 61.1445
      | 61.1725
      | 61.2012
      | 61.2311
      | 61.2635
      | 61.3000
      | 61.3382
      | 61.3767
      | 61.4132
      | 61.4460
      | 61.4749
      | 61.4923
      | 61.5082
      | 61.5257
      | 61.5476
      | 61.5683
      | 61.5924
      | 61.6222
      | 61.6547
      | 61.6888
      | 61.7229
      | 61.7571
      | 61.7915
      | 61.8236
      | 61.8511
      | 61.8759
      | 61.8988
      | 61.9163
      | 61.9323
      | 61.9502
      | 61.9734
      | 61.9976
      | 62.0241
      | 62.0507
      | 62.0773
      | 62.1040
      | 62.1307
      | 62.1575
      | 62.1846
      | 62.2120
      | 62.2402
      | 62.2662
      | 62.2916
      | 62.3151
      | 62.3401
      | 62.3622
      | 62.3835
      | 62.4023
      | 62.4210
      | 62.4393
      | 62.4628
      | 62.4868
      | 62.5121
      | 62.5401
      | 62.5751
      | 62.6159
      | 62.6564
      | 62.6968
      | 62.7369
      | 62.7769
      | 62.8167
      | 62.8564
      | 62.8959
      | 62.9351
      | 62.9742
      | 63.0132
      | 63.0519
      | 63.0905
      | 63.1289
      | 63.1671
      | 63.2051
      | 63.2429
      | 63.2805
      | 63.3180
      | 63.3553
      | 63.3924
      | 63.4293
      | 63.4660
      | 63.5025
      | 63.5389
      | 63.5750
      | 63.6111
      | 63.6469
      | 63.6826
      | 63.7182
      | 63.7535
      | 63.7887
      | 63.8237
      | 63.8585
      | 63.8932
      | 63.9277
      | 63.9621
      | 63.9964
      | 64.0305
      | 64.0645
      | 64.0984
      | 64.1321
      | 64.1657
      | 64.1992
      | 64.2326
      | 64.2658
      | 64.2989
      | 64.3319
      | 64.3647
      | 64.3974
      | 64.4300
      | 64.4625
      | 64.4948
      | 64.5270
      | 64.5534
      | 64.5541
      | 64.5547
      | 64.5552
      | 64.5557
      | 64.5562
      | 64.5566
      | 64.5571
      | 64.5575
      | 64.5579
      | 64.5583
      | 64.5587
      | 64.5592
      | 64.5597
      | 64.5602
      | 64.5607
      | 64.5614
      | 64.5631
      | 64.5676
      | 64.5806
      | 64.5953
      | 64.6086
      | 64.6240
      | 64.6395
      | 64.6549
      | 64.6701
      | 64.6847
      | 64.6973
      | 64.7043
      | 64.7128
      | 64.7255
      | 64.7381
      | 64.7446
      | 64.7515
      | 64.7716
      | 64.7926
      | 64.8160
      | 64.8399
      | 64.8647
      | 64.8914
      | 64.9218
      | 64.9533
      | 64.9838
      | 65.0049
      | 65.0288
      | 65.0540
      | 65.0785
      | 65.1014
      | 65.1247
      | 65.1488
      | 65.1744
      | 65.2033
      | 65.2354
      | 65.2646
      | 65.2912
      | 65.3154
      | 65.3384
      | 65.3576
      | 65.3774
      | 65.3986
      | 65.4180
      | 65.4381
      | 65.4602
      | 65.4820
      | 65.5029
      | 65.5264
      | 65.5513
      | 65.5823
      | 65.6159
      | 65.6518
      | 65.6875
      | 65.7200
      | 65.7516
      | 65.7844
      | 65.8171
      | 65.8497
      | 65.8825
      | 65.9124
      | 65.9460
      | 65.9805
      | 66.0149
      | 66.0491
      | 66.0806
      | 66.1018
      | 66.1086
      | 66.1092
      | 66.1099
      | 66.1106
      | 66.1118
      | 66.1260
      | 66.1534
      | 66.1847
      | 66.2111
      | 66.2334
      | 66.2533
      | 66.2713
      | 66.2894
      | 66.3075
      | 66.3201
      | 66.3273
      | 66.3363
      | 66.3509
      | 66.3749
      | 66.4054
      | 66.4363
      | 66.4683
      | 66.4993
      | 66.5250
      | 66.5454
      | 66.5588
      | 66.5746
      | 66.5970
      | 66.6315
      | 66.6661
      | 66.7007
      | 66.7268
      | 66.7332
      | 66.7340
      | 66.7349
      | 66.7358
      | 66.7368
      | 66.7512
      | 66.7693
      | 66.7868
      | 66.8018
      | 66.8156
      | 66.8260
      | 66.8322
      | 66.8382
      | 66.8495
      | 66.8698
      | 66.8921
      | 66.9177
      | 66.9465
      | 66.9785
      | 67.0108
      | 67.0372
      | 67.0647
      | 67.0944
      | 67.1288
      | 67.1610
      | 67.1912
      | 67.2241
      | 67.2532
      | 67.2806
      | 67.3079
      | 67.3388
      | 67.3737
      | 67.4085
      | 67.4432
      | 67.4777
      | 67.5121
      | 67.5464
      | 67.5739
      | 67.5746
      | 67.5754
      | 67.5762
      | 67.5771
      | 67.5781
      | 67.5791
      | 67.5803
      | 67.5815
      | 67.5828
      | 67.5842
      | 67.5935
      | 67.6143
      | 67.6373
      | 67.6608
      | 67.6851
      | 67.7077
      | 67.7304
      | 67.7532
      | 67.7796
      | 67.8065
      | 67.8348
      | 67.8589
      | 67.8757
      | 67.8881
      | 67.8993
      | 67.9132
      | 67.9288
      | 67.9430
      | 67.9593
      | 67.9755
      | 67.9970
      | 68.0209
      | 68.0457
      | 68.0721
      | 68.0982
      | 68.1240
      | 68.1490
      | 68.1726
      | 68.1917
      | 68.2033
      | 68.2052
      | 68.2072
      | 68.2092
      | 68.2114
      | 68.2137
      | 68.2162
      | 68.2549
      | 68.2925
      | 68.3296
      | 68.3659
      | 68.3981
      | 68.4280
      | 68.4601
      | 68.4960
      | 68.5337
      | 68.5699
      | 68.6031
      | 68.6331
      | 68.6629
      | 68.6891
      | 68.7111
      | 68.7307
      | 68.7496
      | 68.7666
      | 68.7781
      | 68.7862
      | 68.7906
      | 68.7972
      | 68.8095
      | 68.8253
      | 68.8444
      | 68.8713
      | 68.9004
      | 68.9271
      | 68.9526
      | 68.9746
      | 68.9923
      | 69.0168
      | 69.0446
      | 69.0785
      | 69.1117
      | 69.1438
      | 69.1767
      | 69.2085
      | 69.2380
      | 69.2629
      | 69.2843
      | 69.3015
      | 69.3126
      | 69.3313
      | 69.3645
      | 69.4023
      | 69.4399
      | 69.4774
      | 69.5146
      | 69.5517
      | 69.5886
      | 69.6253
      | 69.6615
      | 69.6928
      | 69.7068
      | 69.7085
      | 69.7104
      | 69.7123
      | 69.7144
      | 69.7165
      | 69.7188
      | 69.7211
      | 69.7237
      | 69.7263
      | 69.7347
      | 69.7660
      | 69.8049
      | 69.8437
      | 69.8822
      | 69.9206
      | 69.9588
      | 69.9968
      | 70.0346
      | 70.0723
      | 70.1097
      | 70.1470
      | 70.1841
      | 70.2211
      | 70.2578
      | 70.2943
      | 70.3307
      | 70.3669
      | 70.4030
      | 70.4362
      | 70.4584
      | 70.4748
      | 70.4801
      | 70.4818
      | 70.4836
      | 70.4874
      | 70.5100
      | 70.5358
      | 70.5677
      | 70.6043
      | 70.6346
      | 70.6595
      | 70.6787
      | 70.6974
      | 70.7148
      | 70.7283
      | 70.7424
      | 70.7584
      | 70.7793
      | 70.8022
      | 70.8246
      | 70.8502
      | 70.8783
      | 70.9082
      | 70.9416
      | 70.9699
      | 70.9939
      | 71.0149
      | 71.0328
      | 71.0477
      | 71.0537
      | 71.0585
      | 71.0658
      | 71.0740
      | 71.0849
      | 71.0969
      | 71.1119
      | 71.1290
      | 71.1458
      | 71.1678
      | 71.1917
      | 71.2149
      | 71.2410
      | 71.2652
      | 71.2890
      | 71.3120
      | 71.3324
      | 71.3520
      | 71.3693
      | 71.3862
      | 71.4017
      | 71.4195
      | 71.4375
      | 71.4558
      | 71.4687
      | 71.4854
      | 71.5058
      | 71.5239
      | 71.5418
      | 71.5592
      | 71.5811
      | 71.6027
      | 71.6236
      | 71.6424
      | 71.6617
      | 71.6822
      | 71.7059
      | 71.7318
      | 71.7572
      | 71.7810
      | 71.8073
      | 71.8335
      | 71.8598
      | 71.8861
      | 71.9123
      | 71.9386
      | 71.9649
      | 71.9912
      | 72.0176
      | 72.0442
      | 72.0709
      | 72.0982
      | 72.1264
      | 72.1561
      | 72.1859
      | 72.2156
      | 72.2451
      | 72.2746
      | 72.3040
      | 72.3330
      | 72.3617
      | 72.3896
      | 72.4193
      | 72.4493
      | 72.4799
      | 72.5115
      | 72.5453
      | 72.5770
      | 72.6050
      | 72.6320
      | 72.6574
      | 72.6827
      | 72.7080
      | 72.7332
      | 72.7584
      | 72.7834
      | 72.8079
      | 72.8308
      | 72.8557
      | 72.8798
      | 72.9019
      | 72.9245
      | 72.9483
      | 72.9693
      | 72.9890
      | 73.0111
      | 73.0335
      | 73.0566
      | 73.0812
      | 73.1041
      | 73.1281
      | 73.1549
      | 73.1824
      | 73.2083
      | 73.2342
      | 73.2603
      | 73.2865
      | 73.3132
      | 73.3407
      | 73.3664
      | 73.3921
      | 73.4176
      | 73.4429
      | 73.4671
      | 73.4889
      | 73.5101
      | 73.5298
      | 73.5453
      | 73.5617
      | 73.5802
      | 73.5982
      | 73.6086
      | 73.6232
      | 73.6428
      | 73.6567
      | 73.6745
      | 73.6957
      | 73.7195
      | 73.7438
      | 73.7695
      | 73.7978
      | 73.8269
      | 73.8573
      | 73.8871
      | 73.9158
      | 73.9456
      | 73.9743
      | 74.0007
      | 74.0256
      | 74.0529
      | 74.0801
      | 74.1073
      | 74.1342
      | 74.1603
      | 74.1846
      | 74.2101
      | 74.2382
      | 74.2669
      | 74.2968
      | 74.3256
      | 74.3555
      | 74.3845
      | 74.4117
      | 74.4387
      | 74.4654
      | 74.4913
      | 74.5148
      | 74.5384
      | 74.5621
      | 74.5860
      | 74.6106
      | 74.6366
      | 74.6602
      | 74.6836
      | 74.7065
      | 74.7279
      | 74.7516
      | 74.7751
      | 74.7979
      | 74.8186
      | 74.8403
      | 74.8643
      | 74.8935
      | 74.9265
      | 74.9631
      | 75.0030
      | 75.0410
      | 75.0784
      | 75.1175
      | 75.1517
      | 75.1823
      | 75.2126
      | 75.2422
      | 75.2707
      | 75.2965
      | 75.3202
      | 75.3443
      | 75.3696
      | 75.3973
      | 75.4255
      | 75.4544
      | 75.4845
      | 75.5169
      | 75.5534
      | 75.5914
      | 75.6297
      | 75.6661
      | 75.6990
      | 75.7281
      | 75.7461
      | 75.7626
      | 75.7807
      | 75.8030
      | 75.8242
      | 75.8486
      | 75.8786
      | 75.9111
      | 75.9452
      | 75.9793
      | 76.0135
      | 76.0479
      | 76.0801
      | 76.1078
      | 76.1330
      | 76.1562
      | 76.1743
      | 76.1909
      | 76.2094
      | 76.2330
      | 76.2575
      | 76.2843
      | 76.3112
      | 76.3381
      | 76.3650
      | 76.3920
      | 76.4190
      | 76.4463
      | 76.4740
      | 76.5024
      | 76.5287
      | 76.5544
      | 76.5783
      | 76.6036
      | 76.6261
      | 76.6478
      | 76.6672
      | 76.6865
      | 76.7054
      | 76.7292
      | 76.7535
      | 76.7791
      | 76.8073
      | 76.8423
      | 76.8828
      | 76.9231
      | 76.9633
      | 77.0032
      | 77.0430
      | 77.0827
      | 77.1221
      | 77.1614
      | 77.2005
      | 77.2395
      | 77.2782
      | 77.3168
      | 77.3552
      | 77.3935
      | 77.4315
      | 77.4694
      | 77.5072
      | 77.5447
      | 77.5820
      | 77.6192
      | 77.6562
      | 77.6930
      | 77.7297
      | 77.7661
      | 77.8024
      | 77.8385
      | 77.8745
      | 77.9103
      | 77.9460
      | 77.9815
      | 78.0168
      | 78.0519
      | 78.0869
      | 78.1217
      | 78.1564
      | 78.1909
      | 78.2253
      | 78.2596
      | 78.2937
      | 78.3278
      | 78.3617
      | 78.3954
      | 78.4291
      | 78.4626
      | 78.4960
      | 78.5293
      | 78.5624
      | 78.5955
      | 78.6284
      | 78.6611
      | 78.6938
      | 78.7263
      | 78.7587
      | 78.7910
      | 78.8178
      | 78.8196
      | 78.8214
      | 78.8232
      | 78.8249
      | 78.8266
      | 78.8282
      | 78.8298
      | 78.8315
      | 78.8331
      | 78.8347
      | 78.8364
      | 78.8380
      | 78.8397
      | 78.8414
      | 78.8432
      | 78.8450
      | 78.8480
      | 78.8535
      | 78.8673
      | 78.8826
      | 78.8967
      | 78.9128
      | 78.9289
      | 78.9450
      | 78.9609
      | 78.9762
      | 78.9897
      | 78.9976
      | 79.0070
      | 79.0205
      | 79.0340
      | 79.0414
      | 79.0493
      | 79.0699
      | 79.0914
      | 79.1152
      | 79.1395
      | 79.1646
      | 79.1916
      | 79.2222
      | 79.2537
      | 79.2844
      | 79.3060
      | 79.3303
      | 79.3558
      | 79.3807
      | 79.4040
      | 79.4277
      | 79.4521
      | 79.4781
      | 79.5071
      | 79.5394
      | 79.5688
      | 79.5956
      | 79.6203
      | 79.6437
      | 79.6634
      | 79.6837
      | 79.7054
      | 79.7254
      | 79.7460
      | 79.7686
      | 79.7908
      | 79.8121
      | 79.8361
      | 79.8613
      | 79.8924
      | 79.9261
      | 79.9619
      | 79.9976
      | 80.0302
      | 80.0619
      | 80.0948
      | 80.1276
      | 80.1603
      | 80.1930
      | 80.2231
      | 80.2568
      | 80.2913
      | 80.3257
      | 80.3599
      | 80.3916
      | 80.4132
      | 80.4211
      | 80.4229
      | 80.4248
      | 80.4268
      | 80.4291
      | 80.4441
      | 80.4717
      | 80.5032
      | 80.5299
      | 80.5526
      | 80.5731
      | 80.5917
      | 80.6103
      | 80.6291
      | 80.6424
      | 80.6506
      | 80.6606
      | 80.6759
      | 80.7003
      | 80.7310
      | 80.7620
      | 80.7941
      | 80.8253
      | 80.8513
      | 80.8722
      | 80.8863
      | 80.9028
      | 80.9257
      | 80.9602
      | 80.9948
      | 81.0294
      | 81.0558
      | 81.0633
      | 81.0653
      | 81.0674
      | 81.0695
      | 81.0718
      | 81.0869
      | 81.1057
      | 81.1237
      | 81.1394
      | 81.1540
      | 81.1653
      | 81.1726
      | 81.1796
      | 81.1917
      | 81.2125
      | 81.2353
      | 81.2612
      | 81.2903
      | 81.3224
      | 81.3548
      | 81.3815
      | 81.4092
      | 81.4392
      | 81.4736
      | 81.5058
      | 81.5362
      | 81.5692
      | 81.5985
      | 81.6261
      | 81.6538
      | 81.6848
      | 81.7197
      | 81.7545
      | 81.7892
      | 81.8237
      | 81.8581
      | 81.8924
      | 81.9202
      | 81.9222
      | 81.9242
      | 81.9263
      | 81.9284
      | 81.9306
      | 81.9329
      | 81.9352
      | 81.9377
      | 81.9402
      | 81.9428
      | 81.9531
      | 81.9743
      | 81.9978
      | 82.0217
      | 82.0464
      | 82.0695
      | 82.0926
      | 82.1158
      | 82.1425
      | 82.1698
      | 82.1983
      | 82.2228
      | 82.2403
      | 82.2534
      | 82.2655
      | 82.2802
      | 82.2965
      | 82.3114
      | 82.3285
      | 82.3453
      | 82.3673
      | 82.3916
      | 82.4168
      | 82.4434
      | 82.4699
      | 82.4960
      | 82.5214
      | 82.5454
      | 82.5650
      | 82.5776
      | 82.5806
      | 82.5838
      | 82.5871
      | 82.5904
      | 82.5939
      | 82.5976
      | 82.6362
      | 82.6737
      | 82.7107
      | 82.7469
      | 82.7792
      | 82.8093
      | 82.8415
      | 82.8774
      | 82.9150
      | 82.9512
      | 82.9845
      | 83.0146
      | 83.0445
      | 83.0711
      | 83.0936
      | 83.1137
      | 83.1332
      | 83.1509
      | 83.1632
      | 83.1723
      | 83.1778
      | 83.1854
      | 83.1985
      | 83.2150
      | 83.2347
      | 83.2619
      | 83.2912
      | 83.3182
      | 83.3440
      | 83.3665
      | 83.3849
      | 83.4098
      | 83.4378
      | 83.4718
      | 83.5051
      | 83.5372
      | 83.5702
      | 83.6021
      | 83.6318
      | 83.6571
      | 83.6790
      | 83.6968
      | 83.7088
      | 83.7281
      | 83.7613
      | 83.7990
      | 83.8365
      | 83.8739
      | 83.9111
      | 83.9481
      | 83.9849
      | 84.0216
      | 84.0577
      | 84.0892
      | 84.1039
      | 84.1068
      | 84.1099
      | 84.1130
      | 84.1162
      | 84.1196
      | 84.1230
      | 84.1265
      | 84.1302
      | 84.1340
      | 84.1433
      | 84.1748
      | 84.2136
      | 84.2522
      | 84.2906
      | 84.3289
      | 84.3669
      | 84.4049
      | 84.4426
      | 84.4801
      | 84.5175
      | 84.5547
      | 84.5918
      | 84.6286
      | 84.6653
      | 84.7018
      | 84.7381
      | 84.7743
      | 84.8103
      | 84.8437
      | 84.8663
      | 84.8833
      | 84.8897
      | 84.8926
      | 84.8956
      | 84.9005
      | 84.9235
      | 84.9496
      | 84.9816
      | 85.0182
      | 85.0487
      | 85.0740
      | 85.0937
      | 85.1130
      | 85.1311
      | 85.1453
      | 85.1602
      | 85.1768
      | 85.1982
      | 85.2215
      | 85.2444
      | 85.2703
      | 85.2987
      | 85.3287
      | 85.3622
      | 85.3908
      | 85.4151
      | 85.4366
      | 85.4551
      | 85.4707
      | 85.4778
      | 85.4836
      | 85.4919
      | 85.5011
      | 85.5128
      | 85.5256
      | 85.5413
      | 85.5590
      | 85.5765
      | 85.5989
      | 85.6233
      | 85.6468
      | 85.6732
      | 85.6978
      | 85.7221
      | 85.7454
      | 85.7664
      | 85.7865
      | 85.8044
      | 85.8219
      | 85.8381
      | 85.8566
      | 85.8752
      | 85.8941
      | 85.9077
      | 85.9251
      | 85.9459
      | 85.9646
      | 85.9831
      | 86.0011
      | 86.0235
      | 86.0456
      | 86.0670
      | 86.0863
      | 86.1062
      | 86.1272
      | 86.1513
      | 86.1775
      | 86.2032
      | 86.2275
      | 86.2540
      | 86.2806
      | 86.3071
      | 86.3337
      | 86.3603
      | 86.3868
      | 86.4134
      | 86.4401
      | 86.4668
      | 86.4936
      | 86.5207
      | 86.5482
      | 86.5766
      | 86.6066
      | 86.6365
      | 86.6664
      | 86.6961
      | 86.7258
      | 86.7553
      | 86.7846
      | 86.8135
      | 86.8417
      | 86.8716
      | 86.9017
      | 86.9324
      | 86.9642
      | 86.9980
      | 87.0299
      | 87.0581
      | 87.0854
      | 87.1111
      | 87.1367
      | 87.1623
      | 87.1879
      | 87.2135
      | 87.2388
      | 87.2636
      | 87.2869
      | 87.3122
      | 87.3367
      | 87.3592
      | 87.3821
      | 87.4064
      | 87.4279
      | 87.4481
      | 87.4706
      | 87.4934
      | 87.5169
      | 87.5419
      | 87.5651
      | 87.5896
      | 87.6166
      | 87.6444
      | 87.6706
      | 87.6968
      | 87.7231
      | 87.7497
      | 87.7767
      | 87.8044
      | 87.8304
      | 87.8564
      | 87.8823
      | 87.9078
      | 87.9325
      | 87.9547
      | 87.9763
      | 87.9965
      | 88.0126
      | 88.0296
      | 88.0487
      | 88.0672
      | 88.0784
      | 88.0937
      | 88.1138
      | 88.1285
      | 88.1468
      | 88.1684
      | 88.1926
      | 88.2173
      | 88.2433
      | 88.2718
      | 88.3011
      | 88.3317
      | 88.3617
      | 88.3907
      | 88.4206
      | 88.4496
      | 88.4762
      | 88.5015
      | 88.5290
      | 88.5565
      | 88.5840
      | 88.6111
      | 88.6376
      | 88.6622
      | 88.6880
      | 88.7164
      | 88.7454
      | 88.7754
      | 88.8044
      | 88.8346
      | 88.8638
      | 88.8912
      | 88.9186
      | 88.9456
      | 88.9718
      | 88.9956
      | 89.0196
      | 89.0437
      | 89.0681
      | 89.0930
      | 89.1193
      | 89.1433
      | 89.1671
      | 89.1904
      | 89.2123
      | 89.2365
      | 89.2604
      | 89.2836
      | 89.3048
      | 89.3269
      | 89.3513
      | 89.3808
      | 89.4139
      | 89.4505
      | 89.4904
      | 89.5283
      | 89.5657
      | 89.6048
      | 89.6391
      | 89.6699
      | 89.7004
      | 89.7303
      | 89.7590
      | 89.7853
      | 89.8093
      | 89.8339
      | 89.8595
      | 89.8876
      | 89.9160
      | 89.9452
      | 89.9756
      | 90.0082
      | 90.0447
      | 90.0826
      | 90.1210
      | 90.1575
      | 90.1905
      | 90.2199
      | 90.2385
      | 90.2556
      | 90.2743
      | 90.2972
      | 90.3189
      | 90.3437
      | 90.3740
      | 90.4067
      | 90.4410
      | 90.4752
      | 90.5095
      | 90.5441
      | 90.5765
      | 90.6045
      | 90.6301
      | 90.6538
      | 90.6725
      | 90.6897
      | 90.7089
      | 90.7329
      | 90.7578
      | 90.7850
      | 90.8122
      | 90.8395
      | 90.8668
      | 90.8941
      | 90.9215
      | 90.9492
      | 90.9772
      | 91.0059
      | 91.0326
      | 91.0587
      | 91.0830
      | 91.1087
      | 91.1317
      | 91.1540
      | 91.1739
      | 91.1937
      | 91.2132
      | 91.2375
      | 91.2622
      | 91.2882
      | 91.3167
      | 91.3517
      | 91.3923
      | 91.4326
      | 91.4727
      | 91.5127
      | 91.5525
      | 91.5922
      | 91.6317
      | 91.6710
      | 91.7101
      | 91.7491
      | 91.7879
      | 91.8265
      | 91.8650
      | 91.9032
      | 91.9414
      | 91.9793
      | 92.0170
      | 92.0546
      | 92.0920
      | 92.1292
      | 92.1662
      | 92.2031
      | 92.2397
      | 92.2761
      | 92.3123
      | 92.3483
      | 92.3841
      | 92.4198
      | 92.4553
      | 92.4906
      | 92.5257
      | 92.5608
      | 92.5957
      | 92.6304
      | 92.6651
      | 92.6996
      | 92.7341
      | 92.7684
      | 92.8026
      | 92.8367
      | 92.8707
      | 92.9046
      | 92.9383
      | 92.9719
      | 93.0054
      | 93.0388
      | 93.0721
      | 93.1052
      | 93.1382
      | 93.1711
      | 93.2039
      | 93.2365
      | 93.2690
      | 93.3014
      | 93.3284
      | 93.3312
      | 93.3338
      | 93.3365
      | 93.3390
      | 93.3416
      | 93.3441
      | 93.3466
      | 93.3491
      | 93.3516
      | 93.3541
      | 93.3566
      | 93.3592
      | 93.3617
      | 93.3643
      | 93.3670
      | 93.3697
      | 93.3735
      | 93.3798
      | 93.3942
      | 93.4102
      | 93.4248
      | 93.4415
      | 93.4582
      | 93.4748
      | 93.4913
      | 93.5071
      | 93.5212
      | 93.5299
      | 93.5400
      | 93.5541
      | 93.5682
      | 93.5764
      | 93.5850
      | 93.6061
      | 93.6280
      | 93.6522
      | 93.6769
      | 93.7024
      | 93.7296
      | 93.7604
      | 93.7921
      | 93.8230
      | 93.8450
      | 93.8697
      | 93.8955
      | 93.9207
      | 93.9444
      | 93.9685
      | 93.9933
      | 94.0195
      | 94.0488
      | 94.0811
      | 94.1107
      | 94.1373
      | 94.1608
      | 94.1829
      | 94.2015
      | 94.2205
      | 94.2409
      | 94.2597
      | 94.2790
      | 94.3002
      | 94.3211
      | 94.3412
      | 94.3637
      | 94.3876
      | 94.4173
      | 94.4497
      | 94.4841
      | 94.5185
      | 94.5500
      | 94.5804
      | 94.6122
      | 94.6439
      | 94.6755
      | 94.7073
      | 94.7364
      | 94.7691
      | 94.8028
      | 94.8364
      | 94.8699
      | 94.9007
      | 94.9217
      | 94.9292
      | 94.9308
      | 94.9324
      | 94.9341
      | 94.9360
      | 94.9502
      | 94.9767
      | 95.0072
      | 95.0329
      | 95.0546
      | 95.0742
      | 95.0920
      | 95.1098
      | 95.1278
      | 95.1404
      | 95.1479
      | 95.1571
      | 95.1715
      | 95.1948
      | 95.2243
      | 95.2542
      | 95.2852
      | 95.3153
      | 95.3403
      | 95.3603
      | 95.3737
      | 95.3894
      | 95.4113
      | 95.4448
      | 95.4792
      | 95.5137
      | 95.5403
      | 95.5485
      | 95.5513
      | 95.5542
      | 95.5572
      | 95.5602
      | 95.5759
      | 95.5951
      | 95.6136
      | 95.6299
      | 95.6450
      | 95.6570
      | 95.6649
      | 95.6727
      | 95.6854
      | 95.7067
      | 95.7298
      | 95.7561
      | 95.7853
      | 95.8176
      | 95.8502
      | 95.8771
      | 95.9051
      | 95.9353
      | 95.9698
      | 96.0022
      | 96.0328
      | 96.0659
      | 96.0954
      | 96.1233
      | 96.1512
      | 96.1824
      | 96.2173
      | 96.2522
      | 96.2870
      | 96.3216
      | 96.3561
      | 96.3905
      | 96.4185
      | 96.4213
      | 96.4241
      | 96.4270
      | 96.4300
      | 96.4330
      | 96.4360
      | 96.4392
      | 96.4425
      | 96.4458
      | 96.4493
      | 96.4602
      | 96.4818
      | 96.5056
      | 96.5299
      | 96.5549
      | 96.5784
      | 96.6019
      | 96.6255
      | 96.6524
      | 96.6800
      | 96.7087
      | 96.7335
      | 96.7515
      | 96.7653
      | 96.7779
      | 96.7932
      | 96.8100
      | 96.8255
      | 96.8431
      | 96.8604
      | 96.8828
      | 96.9075
      | 96.9330
      | 96.9600
      | 96.9869
      | 97.0135
      | 97.0397
      | 97.0650
      | 97.0882
      | 97.1104
      | 97.1349
      | 97.1601
      | 97.1897
      | 97.2222
      | 97.2542
      | 97.2858
      | 97.3164
      | 97.3482
      | 97.3797
      | 97.4105
      | 97.4403
      | 97.4709
      | 97.4971
      | 97.5204
      | 97.5390
      | 97.5552
      | 97.5696
      | 97.5900
      | 97.6109
      | 97.6333
      | 97.6585
      | 97.6828
      | 97.7082
      | 97.7328
      | 97.7557
      | 97.7779
      | 97.7985
      | 97.8199
      | 97.8436
      | 97.8711
      | 97.9059
      | 97.9418
      | 97.9775
      | 98.0131
      | 98.0485
      | 98.0837
      | 98.1188
      | 98.1537
      | 98.1885
      | 98.2231
      | 98.2576
      | 98.2920
      | 98.3263
      | 98.3604
      | 98.3945
      | 98.4284
      | 98.4621
      | 98.4958
      | 98.5293
      | 98.5628
      | 98.5961
      | 98.6292
      | 98.6623
      | 98.6952
      | 98.7281
      | 98.7608
      | 98.7933
      | 98.8258
      | 98.8581
      | 98.8903
      | 98.9223
      | 98.9542
      | 98.9859
      | 99.0173
      | 99.0483
      | 99.0790
      | 99.1094
      | 99.1394
      | 99.1692
      | 99.1986
      | 99.2276
      | 99.2563
      | 99.2847
      | 99.3127
      | 99.3403
      | 99.3676
      | 99.3946
      | 99.4212
      | 99.4475
      | 99.4734
      | 99.4989
      | 99.5241
      | 99.5490
      | 99.5735
      | 99.5976
      | 99.6213
      | 99.6447
      | 99.6678
      | 99.6904
      | 99.7127
      | 99.7346
      | 99.7562
      | 99.7773
      | 99.7981
      | 99.8184
      | 99.8384
      | 99.8580
      | 99.8772
      | 99.8959
      | 99.9143
      | 99.9321
      | 99.9496
      | 99.9666
      | 99.9833
      | 100.0000
      | ]
      Table=|
      | [19.9694
      | 19.9729
      | 19.9745
      | 19.9718
      | 19.9668
      | 19.9602
      | 19.9537
      | 19.9471
      | 19.9401
      | 19.9354
      | 19.9345
      | 19.9353
      | 19.9375
      | 19.9423
      | 19.9478
      | 19.9526
      | 19.9547
      | 19.9563
      | 19.9563
      | 19.9563
      | 19.9563
      | 19.9563
      | 19.9563
      | 19.9562
      | 19.9560
      | 19.9556
      | 19.9546
      | 19.9551
      | 19.9560
      | 19.9581
      | 19.9595
      | 19.9624
      | 19.9659
      | 19.9705
      | 19.9753
      | 19.9802
      | 19.9827
      | 19.9848
      | 19.9862
      | 19.9857
      | 19.9794
      | 19.9676
      | 19.9559
      | 19.9443
      | 19.9329
      | 19.9215
      | 19.9103
      | 19.8993
      | 19.8883
      | 19.8775
      | 19.8668
      | 19.8562
      | 19.8458
      | 19.8355
      | 19.8253
      | 19.8152
      | 19.8053
      | 19.7955
      | 19.7858
      | 19.7762
      | 19.7668
      | 19.7575
      | 19.7483
      | 19.7393
      | 19.7303
      | 19.7215
      | 19.7128
      | 19.7042
      | 19.6957
      | 19.6873
      | 19.6790
      | 19.6708
      | 19.6628
      | 19.6548
      | 19.6470
      | 19.6392
      | 19.6316
      | 19.6240
      | 19.6164
      | 19.6090
      | 19.6016
      | 19.5943
      | 19.5871
      | 19.5799
      | 19.5728
      | 19.5657
      | 19.5587
      | 19.5518
      | 19.5449
      | 19.5381
      | 19.5313
      | 19.5246
      | 19.5179
      | 19.5768
      | 19.5676
      | 19.5633
      | 19.5804
      | 19.5590
      | 19.5547
      | 19.5113
      | 19.5505
      | 19.5837
      | 19.5463
      | 19.5421
      | 19.5873
      | 19.5380
      | 19.5339
      | 19.5298
      | 19.5904
      | 19.5258
      | 19.5048
      | 19.5218
      | 19.5935
      | 19.5178
      | 19.5139
      | 19.5100
      | 19.5967
      | 19.5061
      | 19.5022
      | 19.5999
      | 19.6034
      | 19.6074
      | 19.6122
      | 19.6169
      | 19.6210
      | 19.6251
      | 19.6301
      | 19.6351
      | 19.6369
      | 19.6384
      | 19.6387
      | 19.6387
      | 19.6383
      | 19.6369
      | 19.6330
      | 19.6283
      | 19.6243
      | 19.6256
      | 19.6256
      | 19.6250
      | 19.6247
      | 19.6252
      | 19.6256
      | 19.6255
      | 19.6247
      | 19.6218
      | 19.6167
      | 19.6136
      | 19.6122
      | 19.6120
      | 19.6124
      | 19.6145
      | 19.6164
      | 19.6177
      | 19.6198
      | 19.6216
      | 19.6226
      | 19.6237
      | 19.6253
      | 19.6256
      | 19.6253
      | 19.6212
      | 19.6153
      | 19.6076
      | 19.5999
      | 19.5946
      | 19.5900
      | 19.5844
      | 19.5790
      | 19.5735
      | 19.5679
      | 19.5643
      | 19.5580
      | 19.5510
      | 19.5441
      | 19.5373
      | 19.5324
      | 19.5543
      | 19.5500
      | 19.5458
      | 19.5576
      | 19.5416
      | 19.5332
      | 19.5374
      | 19.5555
      | 19.5509
      | 19.5493
      | 19.5498
      | 19.5512
      | 19.5534
      | 19.5556
      | 19.5577
      | 19.5614
      | 19.5659
      | 19.5702
      | 19.5735
      | 19.5734
      | 19.5697
      | 19.5656
      | 19.5609
      | 19.5567
      | 19.5557
      | 19.5570
      | 19.5606
      | 19.5635
      | 19.5641
      | 19.5577
      | 19.5511
      | 19.5445
      | 19.5649
      | 19.5605
      | 19.5562
      | 19.5683
      | 19.5519
      | 19.5432
      | 19.5476
      | 19.5706
      | 19.5732
      | 19.5765
      | 19.5801
      | 19.5843
      | 19.5890
      | 19.5938
      | 19.5980
      | 19.5998
      | 19.6009
      | 19.6004
      | 19.5981
      | 19.5939
      | 19.5895
      | 19.5886
      | 19.5870
      | 19.5842
      | 19.5783
      | 19.5740
      | 19.5708
      | 19.5659
      | 19.5634
      | 19.5617
      | 19.5601
      | 19.5565
      | 19.5502
      | 19.5439
      | 19.5377
      | 19.5316
      | 19.5254
      | 19.5594
      | 19.5550
      | 19.5637
      | 19.5507
      | 19.5464
      | 19.5194
      | 19.5421
      | 19.5379
      | 19.5338
      | 19.5652
      | 19.5296
      | 19.5255
      | 19.5215
      | 19.5174
      | 19.5658
      | 19.5662
      | 19.5662
      | 19.5670
      | 19.5678
      | 19.5686
      | 19.5677
      | 19.5665
      | 19.5646
      | 19.5648
      | 19.5676
      | 19.5715
      | 19.5756
      | 19.5792
      | 19.5825
      | 19.5861
      | 19.5893
      | 19.5925
      | 19.5940
      | 19.5945
      | 19.5947
      | 19.5941
      | 19.5936
      | 19.5933
      | 19.5934
      | 19.5941
      | 19.6301
      | 19.6251
      | 19.6202
      | 19.6152
      | 19.5965
      | 19.6104
      | 19.6055
      | 19.6008
      | 19.6222
      | 19.6150
      | 19.6082
      | 19.6019
      | 19.5982
      | 19.5959
      | 19.5923
      | 19.5861
      | 19.5787
      | 19.5723
      | 19.5678
      | 19.5653
      | 19.5628
      | 19.5621
      | 19.5633
      | 19.5654
      | 19.5677
      | 19.5706
      | 19.5746
      | 19.5838
      | 19.5885
      | 19.5926
      | 19.5960
      | 19.5985
      | 19.5978
      | 19.5961
      | 19.5956
      | 19.5956
      | 19.5971
      | 19.6001
      | 19.6006
      | 19.5996
      | 19.5952
      | 19.5911
      | 19.5877
      | 19.5838
      | 19.5805
      | 19.5786
      | 19.5788
      | 19.5804
      | 19.5834
      | 19.5876
      | 19.5902
      | 19.5862
      | 19.5792
      | 19.5723
      | 19.5654
      | 19.5586
      | 19.5519
      | 19.5453
      | 19.5388
      | 19.5326
      | 19.5722
      | 19.5676
      | 19.5631
      | 19.5766
      | 19.5586
      | 19.5542
      | 19.5498
      | 19.5293
      | 19.5454
      | 19.5411
      | 19.5369
      | 19.5326
      | 19.5737
      | 19.5660
      | 19.5583
      | 19.5508
      | 19.5433
      | 19.5359
      | 19.5286
      | 19.5213
      | 19.5141
      | 19.5070
      | 19.5000
      | 19.4931
      | 19.4862
      | 19.4794
      | 19.4727
      | 19.4661
      | 19.4596
      | 19.4530
      | 19.4482
      | 19.4487
      | 19.4654
      | 19.4617
      | 19.4581
      | 19.4508
      | 19.4545
      | 19.4659
      | 19.4650
      | 19.4611
      | 19.4544
      | 19.4513
      | 19.4507
      | 19.4521
      | 19.4537
      | 19.4557
      | 19.4586
      | 19.4613
      | 19.4637
      | 19.4648
      | 19.4651
      | 19.4656
      | 19.4649
      | 19.4631
      | 19.4604
      | 19.4557
      | 19.4537
      | 19.4536
      | 19.4545
      | 19.4564
      | 19.4590
      | 19.4627
      | 19.4665
      | 19.4702
      | 19.4738
      | 19.4773
      | 19.4806
      | 19.4834
      | 19.4857
      | 19.4881
      | 19.4890
      | 19.4892
      | 19.4898
      | 19.4892
      | 19.4893
      | 19.4896
      | 19.4902
      | 19.4916
      | 19.4934
      | 19.4958
      | 19.4983
      | 19.5011
      | 19.5034
      | 19.5057
      | 19.5080
      | 19.5114
      | 19.5141
      | 19.5158
      | 19.5182
      | 19.5206
      | 19.5232
      | 19.5245
      | 19.5259
      | 19.5276
      | 19.5299
      | 19.5321
      | 19.5339
      | 19.5347
      | 19.5347
      | 19.5348
      | 19.5356
      | 19.5354
      | 19.5352
      | 19.5350
      | 19.5349
      | 19.5347
      | 19.5345
      | 19.5344
      | 19.5342
      | 19.5340
      | 19.5337
      | 19.5333
      | 19.5328
      | 19.5318
      | 19.5301
      | 19.5285
      | 19.5268
      | 19.5252
      | 19.5236
      | 19.5221
      | 19.5207
      | 19.5195
      | 19.5186
      | 19.5169
      | 19.5151
      | 19.5130
      | 19.5103
      | 19.5066
      | 19.5038
      | 19.5028
      | 19.5022
      | 19.5023
      | 19.5024
      | 19.5025
      | 19.5026
      | 19.5028
      | 19.5030
      | 19.5034
      | 19.5044
      | 19.5047
      | 19.5053
      | 19.5066
      | 19.5078
      | 19.5085
      | 19.5101
      | 19.5122
      | 19.5135
      | 19.5148
      | 19.5159
      | 19.5164
      | 19.5175
      | 19.5183
      | 19.5181
      | 19.5175
      | 19.5176
      | 19.5177
      | 19.5178
      | 19.5178
      | 19.5176
      | 19.5171
      | 19.5173
      | 19.5175
      | 19.5178
      | 19.5182
      | 19.5190
      | 19.5206
      | 19.5223
      | 19.5245
      | 19.5277
      | 19.5307
      | 19.5333
      | 19.5360
      | 19.5401
      | 19.5436
      | 19.5460
      | 19.5496
      | 19.5525
      | 19.5546
      | 19.5558
      | 19.5569
      | 19.5576
      | 19.5572
      | 19.5565
      | 19.5552
      | 19.5542
      | 19.5537
      | 19.5527
      | 19.5521
      | 19.5525
      | 19.5534
      | 19.5534
      | 19.5535
      | 19.5536
      | 19.5538
      | 19.5543
      | 19.5554
      | 19.5562
      | 19.5559
      | 19.5554
      | 19.5545
      | 19.5539
      | 19.5529
      | 19.5523
      | 19.5525
      | 19.5526
      | 19.5529
      | 19.5536
      | 19.5550
      | 19.5564
      | 19.5578
      | 19.5592
      | 19.5603
      | 19.5609
      | 19.5624
      | 19.5640
      | 19.5657
      | 19.5679
      | 19.5694
      | 19.5710
      | 19.5728
      | 19.5753
      | 19.5775
      | 19.5790
      | 19.5786
      | 19.5765
      | 19.5727
      | 19.5669
      | 19.5622
      | 19.5578
      | 19.5524
      | 19.5495
      | 19.5483
      | 19.5473
      | 19.5465
      | 19.5462
      | 19.5468
      | 19.5482
      | 19.5495
      | 19.5504
      | 19.5504
      | 19.5503
      | 19.5498
      | 19.5489
      | 19.5469
      | 19.5430
      | 19.5382
      | 19.5332
      | 19.5292
      | 19.5269
      | 19.5263
      | 19.5290
      | 19.5321
      | 19.5349
      | 19.5367
      | 19.5387
      | 19.5399
      | 19.5390
      | 19.5370
      | 19.5342
      | 19.5314
      | 19.5286
      | 19.5256
      | 19.5237
      | 19.5236
      | 19.5244
      | 19.5258
      | 19.5286
      | 19.5317
      | 19.5344
      | 19.5358
      | 19.5369
      | 19.5372
      | 19.5376
      | 19.5379
      | 19.5382
      | 19.5385
      | 19.5388
      | 19.5390
      | 19.5391
      | 19.5389
      | 19.5395
      | 19.5402
      | 19.5416
      | 19.5426
      | 19.5444
      | 19.5464
      | 19.5491
      | 19.5518
      | 19.5546
      | 19.5562
      | 19.5575
      | 19.5585
      | 19.5585
      | 19.5556
      | 19.5499
      | 19.5442
      | 19.5386
      | 19.5331
      | 19.5276
      | 19.5221
      | 19.5167
      | 19.5114
      | 19.5061
      | 19.5009
      | 19.4957
      | 19.4906
      | 19.4855
      | 19.4805
      | 19.4755
      | 19.4706
      | 19.4658
      | 19.4610
      | 19.4563
      | 19.4516
      | 19.4470
      | 19.4424
      | 19.4379
      | 19.4335
      | 19.4291
      | 19.4247
      | 19.4204
      | 19.4162
      | 19.4120
      | 19.4078
      | 19.4037
      | 19.3996
      | 19.3956
      | 19.3916
      | 19.3877
      | 19.3838
      | 19.3800
      | 19.3762
      | 19.3724
      | 19.3686
      | 19.3649
      | 19.3612
      | 19.3575
      | 19.3538
      | 19.3502
      | 19.3466
      | 19.3431
      | 19.3395
      | 19.3360
      | 19.3326
      | 19.3291
      | 19.3257
      | 19.3223
      | 19.3633
      | 19.3662
      | 19.3604
      | 19.3575
      | 19.3547
      | 19.3519
      | 19.3685
      | 19.3492
      | 19.3464
      | 19.3437
      | 19.3706
      | 19.3410
      | 19.3384
      | 19.3189
      | 19.3357
      | 19.3331
      | 19.3729
      | 19.3305
      | 19.3279
      | 19.3253
      | 19.3228
      | 19.3749
      | 19.3202
      | 19.3177
      | 19.3769
      | 19.3789
      | 19.3809
      | 19.3831
      | 19.3856
      | 19.3887
      | 19.3916
      | 19.3942
      | 19.3967
      | 19.3999
      | 19.4030
      | 19.4043
      | 19.4054
      | 19.4058
      | 19.4061
      | 19.4062
      | 19.4056
      | 19.4037
      | 19.4014
      | 19.3994
      | 19.4004
      | 19.4007
      | 19.4006
      | 19.4007
      | 19.4012
      | 19.4017
      | 19.4019
      | 19.4017
      | 19.4003
      | 19.3977
      | 19.3962
      | 19.3957
      | 19.3958
      | 19.3963
      | 19.3978
      | 19.3991
      | 19.4001
      | 19.4015
      | 19.4028
      | 19.4036
      | 19.4045
      | 19.4057
      | 19.4061
      | 19.4062
      | 19.4041
      | 19.4010
      | 19.3968
      | 19.3928
      | 19.3900
      | 19.3876
      | 19.3847
      | 19.3818
      | 19.3789
      | 19.3760
      | 19.3741
      | 19.3707
      | 19.3670
      | 19.3633
      | 19.3596
      | 19.3570
      | 19.3721
      | 19.3691
      | 19.3662
      | 19.3576
      | 19.3633
      | 19.3605
      | 19.3743
      | 19.3733
      | 19.3709
      | 19.3702
      | 19.3707
      | 19.3718
      | 19.3734
      | 19.3749
      | 19.3764
      | 19.3789
      | 19.3818
      | 19.3847
      | 19.3870
      | 19.3872
      | 19.3852
      | 19.3831
      | 19.3805
      | 19.3783
      | 19.3779
      | 19.3790
      | 19.3814
      | 19.3834
      | 19.3840
      | 19.3805
      | 19.3768
      | 19.3732
      | 19.3877
      | 19.3846
      | 19.3816
      | 19.3726
      | 19.3786
      | 19.3756
      | 19.3900
      | 19.3917
      | 19.3935
      | 19.3957
      | 19.3982
      | 19.4011
      | 19.4043
      | 19.4075
      | 19.4104
      | 19.4117
      | 19.4126
      | 19.4126
      | 19.4115
      | 19.4092
      | 19.4068
      | 19.4065
      | 19.4058
      | 19.4043
      | 19.4010
      | 19.3987
      | 19.3970
      | 19.3942
      | 19.3929
      | 19.3922
      | 19.3914
      | 19.3894
      | 19.3858
      | 19.3822
      | 19.3786
      | 19.3751
      | 19.3716
      | 19.3681
      | 19.3975
      | 19.3944
      | 19.3912
      | 19.4005
      | 19.3881
      | 19.3850
      | 19.3820
      | 19.3790
      | 19.3760
      | 19.3730
      | 19.3701
      | 19.4017
      | 19.3671
      | 19.4023
      | 19.4029
      | 19.4032
      | 19.4039
      | 19.4047
      | 19.4054
      | 19.4051
      | 19.4046
      | 19.4037
      | 19.4041
      | 19.4062
      | 19.4089
      | 19.4118
      | 19.4144
      | 19.4168
      | 19.4193
      | 19.4216
      | 19.4239
      | 19.4252
      | 19.4257
      | 19.4261
      | 19.4260
      | 19.4260
      | 19.4261
      | 19.4264
      | 19.4271
      | 19.4289
      | 19.4533
      | 19.4496
      | 19.4460
      | 19.4425
      | 19.4389
      | 19.4354
      | 19.4319
      | 19.4486
      | 19.4444
      | 19.4404
      | 19.4367
      | 19.4347
      | 19.4335
      | 19.4315
      | 19.4280
      | 19.4236
      | 19.4198
      | 19.4173
      | 19.4160
      | 19.4147
      | 19.4145
      | 19.4156
      | 19.4172
      | 19.4190
      | 19.4212
      | 19.4241
      | 19.4274
      | 19.4309
      | 19.4343
      | 19.4373
      | 19.4398
      | 19.4417
      | 19.4416
      | 19.4408
      | 19.4408
      | 19.4411
      | 19.4424
      | 19.4446
      | 19.4453
      | 19.4450
      | 19.4424
      | 19.4401
      | 19.4382
      | 19.4360
      | 19.4342
      | 19.4332
      | 19.4337
      | 19.4350
      | 19.4373
      | 19.4404
      | 19.4425
      | 19.4402
      | 19.4359
      | 19.4317
      | 19.4276
      | 19.4235
      | 19.4194
      | 19.4154
      | 19.4115
      | 19.4077
      | 19.4390
      | 19.4355
      | 19.4320
      | 19.4285
      | 19.4251
      | 19.4424
      | 19.4217
      | 19.4183
      | 19.4150
      | 19.4117
      | 19.4084
      | 19.4408
      | 19.4361
      | 19.4314
      | 19.4268
      | 19.4222
      | 19.4177
      | 19.4132
      | 19.4087
      | 19.4043
      | 19.3999
      | 19.3956
      | 19.3913
      | 19.3871
      | 19.3829
      | 19.3787
      | 19.3746
      | 19.3705
      | 19.3665
      | 19.3636
      | 19.3642
      | 19.3749
      | 19.3780
      | 19.3660
      | 19.3719
      | 19.3690
      | 19.3786
      | 19.3783
      | 19.3761
      | 19.3718
      | 19.3701
      | 19.3700
      | 19.3714
      | 19.3728
      | 19.3745
      | 19.3769
      | 19.3792
      | 19.3812
      | 19.3823
      | 19.3829
      | 19.3836
      | 19.3834
      | 19.3825
      | 19.3810
      | 19.3781
      | 19.3771
      | 19.3774
      | 19.3784
      | 19.3801
      | 19.3823
      | 19.3853
      | 19.3884
      | 19.3915
      | 19.3945
      | 19.3973
      | 19.4000
      | 19.4024
      | 19.4044
      | 19.4065
      | 19.4075
      | 19.4080
      | 19.4088
      | 19.4087
      | 19.4092
      | 19.4097
      | 19.4105
      | 19.4120
      | 19.4136
      | 19.4156
      | 19.4178
      | 19.4202
      | 19.4223
      | 19.4243
      | 19.4263
      | 19.4291
      | 19.4314
      | 19.4330
      | 19.4351
      | 19.4373
      | 19.4395
      | 19.4408
      | 19.4422
      | 19.4438
      | 19.4459
      | 19.4478
      | 19.4495
      | 19.4504
      | 19.4508
      | 19.4513
      | 19.4522
      | 19.4524
      | 19.4527
      | 19.4529
      | 19.4532
      | 19.4534
      | 19.4537
      | 19.4539
      | 19.4541
      | 19.4544
      | 19.4545
      | 19.4546
      | 19.4546
      | 19.4543
      | 19.4534
      | 19.4525
      | 19.4517
      | 19.4508
      | 19.4500
      | 19.4493
      | 19.4486
      | 19.4480
      | 19.4477
      | 19.4468
      | 19.4458
      | 19.4446
      | 19.4430
      | 19.4405
      | 19.4388
      | 19.4384
      | 19.4383
      | 19.4387
      | 19.4391
      | 19.4395
      | 19.4399
      | 19.4404
      | 19.4409
      | 19.4416
      | 19.4426
      | 19.4432
      | 19.4440
      | 19.4453
      | 19.4465
      | 19.4474
      | 19.4489
      | 19.4508
      | 19.4522
      | 19.4535
      | 19.4547
      | 19.4554
      | 19.4566
      | 19.4575
      | 19.4576
      | 19.4575
      | 19.4579
      | 19.4583
      | 19.4587
      | 19.4589
      | 19.4591
      | 19.4590
      | 19.4595
      | 19.4600
      | 19.4605
      | 19.4611
      | 19.4620
      | 19.4635
      | 19.4652
      | 19.4672
      | 19.4700
      | 19.4727
      | 19.4751
      | 19.4775
      | 19.4811
      | 19.4842
      | 19.4864
      | 19.4896
      | 19.4922
      | 19.4941
      | 19.4954
      | 19.4966
      | 19.4974
      | 19.4973
      | 19.4970
      | 19.4963
      | 19.4958
      | 19.4956
      | 19.4951
      | 19.4949
      | 19.4955
      | 19.4965
      | 19.4968
      | 19.4971
      | 19.4974
      | 19.4978
      | 19.4985
      | 19.4997
      | 19.5006
      | 19.5006
      | 19.5005
      | 19.5000
      | 19.4998
      | 19.4993
      | 19.4990
      | 19.4994
      | 19.4998
      | 19.5003
      | 19.5010
      | 19.5025
      | 19.5039
      | 19.5053
      | 19.5066
      | 19.5078
      | 19.5086
      | 19.5100
      | 19.5116
      | 19.5132
      | 19.5153
      | 19.5167
      | 19.5183
      | 19.5201
      | 19.5223
      | 19.5244
      | 19.5259
      | 19.5258
      | 19.5243
      | 19.5214
      | 19.5169
      | 19.5133
      | 19.5099
      | 19.5057
      | 19.5036
      | 19.5029
      | 19.5022
      | 19.5018
      | 19.5018
      | 19.5025
      | 19.5039
      | 19.5052
      | 19.5062
      | 19.5064
      | 19.5065
      | 19.5064
      | 19.5058
      | 19.5044
      | 19.5014
      | 19.4976
      | 19.4936
      | 19.4905
      | 19.4888
      | 19.4884
      | 19.4910
      | 19.4939
      | 19.4964
      | 19.4981
      | 19.5001
      | 19.5013
      | 19.5007
      | 19.4992
      | 19.4971
      | 19.4949
      | 19.4927
      | 19.4904
      | 19.4890
      | 19.4891
      | 19.4899
      | 19.4913
      | 19.4939
      | 19.4968
      | 19.4993
      | 19.5007
      | 19.5018
      | 19.5023
      | 19.5027
      | 19.5032
      | 19.5037
      | 19.5041
      | 19.5045
      | 19.5049
      | 19.5051
      | 19.5051
      | 19.5058
      | 19.5066
      | 19.5080
      | 19.5090
      | 19.5107
      | 19.5126
      | 19.5151
      | 19.5176
      | 19.5203
      | 19.5218
      | 19.5231
      | 19.5241
      | 19.5243
      | 19.5220
      | 19.5172
      | 19.5125
      | 19.5078
      | 19.5031
      | 19.4985
      | 19.4939
      | 19.4894
      | 19.4849
      | 19.4804
      | 19.4760
      | 19.4717
      | 19.4673
      | 19.4630
      | 19.4588
      | 19.4546
      | 19.4504
      | 19.4463
      | 19.4422
      | 19.4382
      | 19.4342
      | 19.4303
      | 19.4264
      | 19.4225
      | 19.4187
      | 19.4149
      | 19.4112
      | 19.4075
      | 19.4038
      | 19.4002
      | 19.3966
      | 19.3931
      | 19.3895
      | 19.3861
      | 19.3826
      | 19.3792
      | 19.3759
      | 19.3725
      | 19.3692
      | 19.3659
      | 19.3626
      | 19.3593
      | 19.3561
      | 19.3529
      | 19.3497
      | 19.3465
      | 19.3433
      | 19.3402
      | 19.3371
      | 19.3340
      | 19.3309
      | 19.3279
      | 19.3249
      | 19.3219
      | 19.3641
      | 19.3612
      | 19.3670
      | 19.3583
      | 19.3555
      | 19.3526
      | 19.3189
      | 19.3498
      | 19.3470
      | 19.3443
      | 19.3693
      | 19.3415
      | 19.3388
      | 19.3361
      | 19.3335
      | 19.3308
      | 19.3282
      | 19.3256
      | 19.3713
      | 19.3230
      | 19.3204
      | 19.3178
      | 19.3736
      | 19.3755
      | 19.3775
      | 19.3795
      | 19.3815
      | 19.3837
      | 19.3861
      | 19.3891
      | 19.3920
      | 19.3945
      | 19.3971
      | 19.4002
      | 19.4033
      | 19.4046
      | 19.4057
      | 19.4062
      | 19.4066
      | 19.4067
      | 19.4063
      | 19.4047
      | 19.4027
      | 19.4010
      | 19.4021
      | 19.4024
      | 19.4024
      | 19.4026
      | 19.4032
      | 19.4038
      | 19.4041
      | 19.4040
      | 19.4029
      | 19.4006
      | 19.3993
      | 19.3989
      | 19.3991
      | 19.3997
      | 19.4011
      | 19.4025
      | 19.4035
      | 19.4050
      | 19.4063
      | 19.4071
      | 19.4081
      | 19.4092
      | 19.4097
      | 19.4099
      | 19.4081
      | 19.4053
      | 19.4015
      | 19.3978
      | 19.3954
      | 19.3932
      | 19.3906
      | 19.3880
      | 19.3854
      | 19.3827
      | 19.3811
      | 19.3780
      | 19.3746
      | 19.3712
      | 19.3678
      | 19.3655
      | 19.3810
      | 19.3780
      | 19.3662
      | 19.3750
      | 19.3720
      | 19.3690
      | 19.3832
      | 19.3824
      | 19.3802
      | 19.3797
      | 19.3803
      | 19.3814
      | 19.3830
      | 19.3845
      | 19.3860
      | 19.3885
      | 19.3915
      | 19.3944
      | 19.3966
      | 19.3969
      | 19.3951
      | 19.3932
      | 19.3909
      | 19.3889
      | 19.3886
      | 19.3897
      | 19.3921
      | 19.3942
      | 19.3948
      | 19.3915
      | 19.3882
      | 19.3848
      | 19.4000
      | 19.3968
      | 19.3844
      | 19.3936
      | 19.3905
      | 19.3874
      | 19.4023
      | 19.4040
      | 19.4059
      | 19.4081
      | 19.4106
      | 19.4135
      | 19.4168
      | 19.4201
      | 19.4230
      | 19.4244
      | 19.4253
      | 19.4253
      | 19.4244
      | 19.4223
      | 19.4201
      | 19.4199
      | 19.4193
      | 19.4180
      | 19.4150
      | 19.4127
      | 19.4112
      | 19.4087
      | 19.4075
      | 19.4068
      | 19.4062
      | 19.4044
      | 19.4010
      | 19.3976
      | 19.3943
      | 19.3909
      | 19.3876
      | 19.3844
      | 19.4155
      | 19.4122
      | 19.4089
      | 19.4056
      | 19.4024
      | 19.3992
      | 19.3960
      | 19.4186
      | 19.3928
      | 19.3897
      | 19.3866
      | 19.3835
      | 19.4198
      | 19.4205
      | 19.4211
      | 19.4215
      | 19.4223
      | 19.4231
      | 19.4239
      | 19.4237
      | 19.4234
      | 19.4226
      | 19.4230
      | 19.4251
      | 19.4279
      | 19.4309
      | 19.4335
      | 19.4359
      | 19.4386
      | 19.4409
      | 19.4432
      | 19.4445
      | 19.4452
      | 19.4456
      | 19.4456
      | 19.4457
      | 19.4458
      | 19.4462
      | 19.4469
      | 19.4488
      | 19.4667
      | 19.4743
      | 19.4592
      | 19.4555
      | 19.4519
      | 19.4698
      | 19.4658
      | 19.4620
      | 19.4585
      | 19.4566
      | 19.4555
      | 19.4536
      | 19.4502
      | 19.4460
      | 19.4424
      | 19.4399
      | 19.4387
      | 19.4375
      | 19.4374
      | 19.4385
      | 19.4402
      | 19.4421
      | 19.4443
      | 19.4473
      | 19.4507
      | 19.4544
      | 19.4579
      | 19.4610
      | 19.4636
      | 19.4655
      | 19.4655
      | 19.4648
      | 19.4648
      | 19.4652
      | 19.4665
      | 19.4688
      | 19.4695
      | 19.4692
      | 19.4667
      | 19.4645
      | 19.4627
      | 19.4605
      | 19.4588
      | 19.4578
      | 19.4583
      | 19.4597
      | 19.4620
      | 19.4653
      | 19.4674
      | 19.4651
      | 19.4610
      | 19.4568
      | 19.4527
      | 19.4487
      | 19.4447
      | 19.4407
      | 19.4368
      | 19.4331
      | 19.4312
      | 19.4517
      | 19.4481
      | 19.4445
      | 19.4665
      | 19.4409
      | 19.4374
      | 19.4339
      | 19.4700
      | 19.4685
      | 19.4638
      | 19.4592
      | 19.4546
      | 19.4501
      | 19.4456
      | 19.4411
      | 19.4367
      | 19.4323
      | 19.4279
      | 19.4236
      | 19.4194
      | 19.4151
      | 19.4110
      | 19.4068
      | 19.4027
      | 19.3987
      | 19.3946
      | 19.3917
      | 19.3924
      | 19.3943
      | 19.4039
      | 19.4006
      | 19.3974
      | 19.4071
      | 19.4078
      | 19.4076
      | 19.4053
      | 19.4011
      | 19.3993
      | 19.3993
      | 19.4007
      | 19.4022
      | 19.4040
      | 19.4065
      | 19.4089
      | 19.4110
      | 19.4121
      | 19.4128
      | 19.4135
      | 19.4134
      | 19.4125
      | 19.4110
      | 19.4081
      | 19.4071
      | 19.4074
      | 19.4085
      | 19.4102
      | 19.4125
      | 19.4158
      | 19.4191
      | 19.4223
      | 19.4255
      | 19.4285
      | 19.4314
      | 19.4338
      | 19.4359
      | 19.4381
      | 19.4392
      | 19.4398
      | 19.4406
      | 19.4405
      | 19.4410
      | 19.4416
      | 19.4425
      | 19.4440
      | 19.4457
      | 19.4478
      | 19.4501
      | 19.4526
      | 19.4548
      | 19.4569
      | 19.4589
      | 19.4619
      | 19.4643
      | 19.4660
      | 19.4682
      | 19.4704
      | 19.4728
      | 19.4742
      | 19.4756
      | 19.4773
      | 19.4794
      | 19.4815
      | 19.4832
      | 19.4842
      | 19.4846
      | 19.4852
      | 19.4861
      | 19.4864
      | 19.4867
      | 19.4870
      | 19.4872
      | 19.4875
      | 19.4878
      | 19.4881
      | 19.4884
      | 19.4886
      | 19.4888
      | 19.4890
      | 19.4889
      | 19.4886
      | 19.4878
      | 19.4869
      | 19.4861
      | 19.4853
      | 19.4845
      | 19.4837
      | 19.4831
      | 19.4825
      | 19.4822
      | 19.4813
      | 19.4803
      | 19.4791
      | 19.4775
      | 19.4750
      | 19.4733
      | 19.4729
      | 19.4729
      | 19.4733
      | 19.4737
      | 19.4742
      | 19.4746
      | 19.4751
      | 19.4757
      | 19.4764
      | 19.4775
      | 19.4781
      | 19.4789
      | 19.4803
      | 19.4816
      | 19.4825
      | 19.4841
      | 19.4861
      | 19.4875
      | 19.4889
      | 19.4901
      | 19.4909
      | 19.4922
      | 19.4931
      | 19.4933
      | 19.4932
      | 19.4936
      | 19.4940
      | 19.4944
      | 19.4947
      | 19.4949
      | 19.4949
      | 19.4954
      | 19.4959
      | 19.4964
      | 19.4971
      | 19.4980
      | 19.4996
      | 19.5014
      | 19.5035
      | 19.5064
      | 19.5093
      | 19.5117
      | 19.5143
      | 19.5180
      | 19.5212
      | 19.5235
      | 19.5269
      | 19.5296
      | 19.5316
      | 19.5330
      | 19.5342
      | 19.5350
      | 19.5350
      | 19.5348
      | 19.5340
      | 19.5335
      | 19.5334
      | 19.5328
      | 19.5327
      | 19.5333
      | 19.5343
      | 19.5346
      | 19.5350
      | 19.5353
      | 19.5358
      | 19.5365
      | 19.5378
      | 19.5387
      | 19.5387
      | 19.5386
      | 19.5381
      | 19.5380
      | 19.5374
      | 19.5372
      | 19.5376
      | 19.5380
      | 19.5385
      | 19.5393
      | 19.5408
      | 19.5423
      | 19.5437
      | 19.5451
      | 19.5463
      | 19.5471
      | 19.5487
      | 19.5502
      | 19.5520
      | 19.5541
      | 19.5556
      | 19.5572
      | 19.5591
      | 19.5614
      | 19.5636
      | 19.5651
      | 19.5650
      | 19.5635
      | 19.5606
      | 19.5560
      | 19.5523
      | 19.5488
      | 19.5446
      | 19.5424
      | 19.5416
      | 19.5410
      | 19.5405
      | 19.5405
      | 19.5413
      | 19.5427
      | 19.5440
      | 19.5451
      | 19.5453
      | 19.5454
      | 19.5452
      | 19.5447
      | 19.5432
      | 19.5401
      | 19.5362
      | 19.5322
      | 19.5289
      | 19.5272
      | 19.5268
      | 19.5295
      | 19.5324
      | 19.5351
      | 19.5369
      | 19.5389
      | 19.5401
      | 19.5395
      | 19.5380
      | 19.5358
      | 19.5336
      | 19.5313
      | 19.5289
      | 19.5274
      | 19.5275
      | 19.5284
      | 19.5298
      | 19.5325
      | 19.5355
      | 19.5381
      | 19.5396
      | 19.5407
      | 19.5412
      | 19.5417
      | 19.5421
      | 19.5426
      | 19.5431
      | 19.5435
      | 19.5438
      | 19.5441
      | 19.5440
      | 19.5447
      | 19.5455
      | 19.5469
      | 19.5480
      | 19.5497
      | 19.5517
      | 19.5543
      | 19.5569
      | 19.5597
      | 19.5612
      | 19.5626
      | 19.5636
      | 19.5638
      | 19.5614
      | 19.5565
      | 19.5516
      | 19.5467
      | 19.5419
      | 19.5372
      | 19.5324
      | 19.5277
      | 19.5231
      | 19.5185
      | 19.5139
      | 19.5094
      | 19.5049
      | 19.5005
      | 19.4961
      | 19.4917
      | 19.4874
      | 19.4831
      | 19.4789
      | 19.4747
      | 19.4705
      | 19.4664
      | 19.4624
      | 19.4584
      | 19.4544
      | 19.4505
      | 19.4466
      | 19.4428
      | 19.4389
      | 19.4352
      | 19.4314
      | 19.4277
      | 19.4241
      | 19.4204
      | 19.4169
      | 19.4133
      | 19.4098
      | 19.4063
      | 19.4028
      | 19.3993
      | 19.3959
      | 19.3925
      | 19.3891
      | 19.3857
      | 19.3824
      | 19.3791
      | 19.3758
      | 19.3725
      | 19.3692
      | 19.3660
      | 19.3627
      | 19.3595
      | 19.3564
      | 19.3532
      | 19.3501
      | 19.3969
      | 19.3937
      | 19.3906
      | 19.3874
      | 19.3843
      | 19.3812
      | 19.4033
      | 19.3782
      | 19.3752
      | 19.3722
      | 19.3692
      | 19.3662
      | 19.3633
      | 19.3604
      | 19.3575
      | 19.3546
      | 19.3518
      | 19.3490
      | 19.4057
      | 19.4078
      | 19.4102
      | 19.4123
      | 19.4143
      | 19.4164
      | 19.4186
      | 19.4209
      | 19.4234
      | 19.4267
      | 19.4298
      | 19.4324
      | 19.4351
      | 19.4385
      | 19.4418
      | 19.4432
      | 19.4443
      | 19.4448
      | 19.4452
      | 19.4454
      | 19.4450
      | 19.4433
      | 19.4412
      | 19.4394
      | 19.4405
      | 19.4409
      | 19.4409
      | 19.4411
      | 19.4417
      | 19.4422
      | 19.4426
      | 19.4424
      | 19.4413
      | 19.4389
      | 19.4375
      | 19.4371
      | 19.4373
      | 19.4379
      | 19.4394
      | 19.4408
      | 19.4418
      | 19.4434
      | 19.4447
      | 19.4456
      | 19.4465
      | 19.4477
      | 19.4482
      | 19.4484
      | 19.4464
      | 19.4435
      | 19.4395
      | 19.4356
      | 19.4330
      | 19.4307
      | 19.4279
      | 19.4251
      | 19.4224
      | 19.4195
      | 19.4177
      | 19.4145
      | 19.4109
      | 19.4072
      | 19.4036
      | 19.4011
      | 19.4018
      | 19.4181
      | 19.4114
      | 19.4081
      | 19.4049
      | 19.4204
      | 19.4195
      | 19.4171
      | 19.4165
      | 19.4171
      | 19.4182
      | 19.4198
      | 19.4214
      | 19.4230
      | 19.4256
      | 19.4288
      | 19.4319
      | 19.4342
      | 19.4344
      | 19.4325
      | 19.4304
      | 19.4279
      | 19.4257
      | 19.4254
      | 19.4265
      | 19.4290
      | 19.4311
      | 19.4317
      | 19.4282
      | 19.4246
      | 19.4210
      | 19.4205
      | 19.4376
      | 19.4340
      | 19.4306
      | 19.4271
      | 19.4237
      | 19.4400
      | 19.4417
      | 19.4436
      | 19.4460
      | 19.4486
      | 19.4517
      | 19.4552
      | 19.4587
      | 19.4618
      | 19.4632
      | 19.4641
      | 19.4641
      | 19.4630
      | 19.4607
      | 19.4583
      | 19.4580
      | 19.4574
      | 19.4559
      | 19.4526
      | 19.4502
      | 19.4485
      | 19.4457
      | 19.4444
      | 19.4436
      | 19.4429
      | 19.4408
      | 19.4372
      | 19.4336
      | 19.4300
      | 19.4264
      | 19.4228
      | 19.4193
      | 19.4390
      | 19.4461
      | 19.4497
      | 19.4320
      | 19.4534
      | 19.4285
      | 19.4251
      | 19.4217
      | 19.4183
      | 19.4566
      | 19.4579
      | 19.4586
      | 19.4591
      | 19.4595
      | 19.4602
      | 19.4610
      | 19.4618
      | 19.4615
      | 19.4611
      | 19.4602
      | 19.4605
      | 19.4627
      | 19.4657
      | 19.4688
      | 19.4716
      | 19.4741
      | 19.4768
      | 19.4792
      | 19.4817
      | 19.4830
      | 19.4836
      | 19.4840
      | 19.4839
      | 19.4839
      | 19.4840
      | 19.4843
      | 19.4850
      | 19.4869
      | 19.4902
      | 19.4941
      | 19.4981
      | 19.5021
      | 19.5062
      | 19.5103
      | 19.5144
      | 19.5097
      | 19.5054
      | 19.5014
      | 19.4977
      | 19.4957
      | 19.4945
      | 19.4925
      | 19.4888
      | 19.4844
      | 19.4805
      | 19.4780
      | 19.4766
      | 19.4753
      | 19.4752
      | 19.4763
      | 19.4780
      | 19.4799
      | 19.4822
      | 19.4854
      | 19.4890
      | 19.4929
      | 19.4967
      | 19.4999
      | 19.5026
      | 19.5047
      | 19.5046
      | 19.5037
      | 19.5037
      | 19.5041
      | 19.5054
      | 19.5078
      | 19.5085
      | 19.5081
      | 19.5055
      | 19.5031
      | 19.5012
      | 19.4989
      | 19.4970
      | 19.4960
      | 19.4965
      | 19.4979
      | 19.5003
      | 19.5037
      | 19.5059
      | 19.5035
      | 19.4991
      | 19.4948
      | 19.4905
      | 19.4863
      | 19.4821
      | 19.4779
      | 19.4738
      | 19.4699
      | 19.4679
      | 19.4707
      | 19.4745
      | 19.4783
      | 19.4822
      | 19.4861
      | 19.4900
      | 19.4940
      | 19.4980
      | 19.5020
      | 19.5060
      | 19.5098
      | 19.5081
      | 19.5033
      | 19.4985
      | 19.4937
      | 19.4889
      | 19.4842
      | 19.4796
      | 19.4749
      | 19.4704
      | 19.4658
      | 19.4613
      | 19.4569
      | 19.4525
      | 19.4481
      | 19.4438
      | 19.4395
      | 19.4352
      | 19.4310
      | 19.4280
      | 19.4286
      | 19.4306
      | 19.4340
      | 19.4375
      | 19.4410
      | 19.4445
      | 19.4452
      | 19.4449
      | 19.4425
      | 19.4381
      | 19.4363
      | 19.4362
      | 19.4377
      | 19.4392
      | 19.4411
      | 19.4437
      | 19.4462
      | 19.4484
      | 19.4496
      | 19.4502
      | 19.4510
      | 19.4508
      | 19.4498
      | 19.4482
      | 19.4452
      | 19.4441
      | 19.4444
      | 19.4455
      | 19.4473
      | 19.4497
      | 19.4532
      | 19.4568
      | 19.4602
      | 19.4636
      | 19.4668
      | 19.4698
      | 19.4724
      | 19.4746
      | 19.4768
      | 19.4779
      | 19.4785
      | 19.4793
      | 19.4792
      | 19.4797
      | 19.4803
      | 19.4811
      | 19.4827
      | 19.4844
      | 19.4867
      | 19.4890
      | 19.4917
      | 19.4939
      | 19.4961
      | 19.4982
      | 19.5013
      | 19.5039
      | 19.5056
      | 19.5079
      | 19.5102
      | 19.5126
      | 19.5140
      | 19.5155
      | 19.5172
      | 19.5194
      | 19.5215
      | 19.5234
      | 19.5244
      | 19.5247
      | 19.5252
      | 19.5262
      | 19.5264
      | 19.5267
      | 19.5270
      | 19.5272
      | 19.5275
      | 19.5277
      | 19.5280
      | 19.5282
      | 19.5284
      | 19.5286
      | 19.5287
      | 19.5286
      | 19.5283
      | 19.5273
      | 19.5264
      | 19.5254
      | 19.5245
      | 19.5237
      | 19.5229
      | 19.5221
      | 19.5215
      | 19.5212
      | 19.5202
      | 19.5191
      | 19.5178
      | 19.5160
      | 19.5134
      | 19.5116
      | 19.5111
      | 19.5110
      | 19.5114
      | 19.5118
      | 19.5122
      | 19.5127
      | 19.5131
      | 19.5136
      | 19.5143
      | 19.5155
      | 19.5160
      | 19.5168
      | 19.5182
      | 19.5195
      | 19.5204
      | 19.5221
      | 19.5241
      | 19.5255
      | 19.5269
      | 19.5281
      | 19.5288
      | 19.5301
      | 19.5311
      | 19.5312
      | 19.5310
      | 19.5314
      | 19.5318
      | 19.5321
      | 19.5324
      | 19.5326
      | 19.5324
      | 19.5329
      | 19.5334
      | 19.5339
      | 19.5345
      | 19.5354
      | 19.5370
      | 19.5388
      | 19.5410
      | 19.5440
      | 19.5469
      | 19.5494
      | 19.5521
      | 19.5560
      | 19.5593
      | 19.5617
      | 19.5652
      | 19.5680
      | 19.5700
      | 19.5714
      | 19.5726
      | 19.5734
      | 19.5733
      | 19.5730
      | 19.5721
      | 19.5715
      | 19.5713
      | 19.5707
      | 19.5705
      | 19.5711
      | 19.5721
      | 19.5724
      | 19.5726
      | 19.5730
      | 19.5734
      | 19.5740
      | 19.5753
      | 19.5762
      | 19.5762
      | 19.5760
      | 19.5754
      | 19.5752
      | 19.5745
      | 19.5742
      | 19.5746
      | 19.5749
      | 19.5754
      | 19.5762
      | 19.5777
      | 19.5791
      | 19.5806
      | 19.5819
      | 19.5832
      | 19.5839
      | 19.5855
      | 19.5870
      | 19.5888
      | 19.5909
      | 19.5924
      | 19.5941
      | 19.5959
      | 19.5983
      | 19.6004
      | 19.6020
      | 19.6018
      | 19.6002
      | 19.5971
      | 19.5923
      | 19.5885
      | 19.5848
      | 19.5804
      | 19.5781
      | 19.5772
      | 19.5765
      | 19.5760
      | 19.5759
      | 19.5766
      | 19.5781
      | 19.5794
      | 19.5804
      | 19.5805
      | 19.5806
      | 19.5804
      | 19.5797
      | 19.5781
      | 19.5749
      | 19.5708
      | 19.5666
      | 19.5632
      | 19.5613
      | 19.5609
      | 19.5636
      | 19.5667
      | 19.5694
      | 19.5712
      | 19.5732
      | 19.5744
      | 19.5737
      | 19.5721
      | 19.5698
      | 19.5674
      | 19.5651
      | 19.5625
      | 19.5609
      | 19.5610
      | 19.5618
      | 19.5632
      | 19.5660
      | 19.5690
      | 19.5717
      | 19.5731
      | 19.5742
      | 19.5747
      | 19.5751
      | 19.5755
      | 19.5759
      | 19.5763
      | 19.5767
      | 19.5770
      | 19.5772
      | 19.5771
      | 19.5777
      | 19.5785
      | 19.5799
      | 19.5809
      | 19.5826
      | 19.5846
      | 19.5873
      | 19.5899
      | 19.5927
      | 19.5942
      | 19.5956
      | 19.5966
      | 19.5967
      | 19.5942
      | 19.5891
      | 19.5841
      | 19.5791
      | 19.5741
      | 19.5692
      | 19.5643
      | 19.5595
      | 19.5547
      | 19.5499
      | 19.5452
      | 19.5405
      | 19.5359
      | 19.5313
      | 19.5268
      | 19.5223
      | 19.5178
      | 19.5134
      | 19.5090
      | 19.5047
      | 19.5004
      | 19.4962
      | 19.4920
      | 19.4879
      | 19.4838
      | 19.4798
      | 19.4758
      | 19.4718
      | 19.4678
      | 19.4639
      | 19.4601
      | 19.4563
      | 19.4525
      | 19.4487
      | 19.4451
      | 19.4414
      | 19.4378
      | 19.4341
      | 19.4305
      | 19.4270
      | 19.4234
      | 19.4199
      | 19.4164
      | 19.4129
      | 19.4095
      | 19.4061
      | 19.4026
      | 19.3993
      | 19.3959
      | 19.3925
      | 19.3892
      | 19.3859
      | 19.3826
      | 19.3794
      | 19.3762
      | 19.3750
      | 19.3780
      | 19.3810
      | 19.3841
      | 19.3872
      | 19.3904
      | 19.3935
      | 19.3967
      | 19.3999
      | 19.4031
      | 19.4064
      | 19.4097
      | 19.4130
      | 19.4163
      | 19.4197
      | 19.4231
      | 19.4265
      | 19.4299
      | 19.4333
      | 19.4358
      | 19.4380
      | 19.4405
      | 19.4426
      | 19.4447
      | 19.4469
      | 19.4491
      | 19.4514
      | 19.4541
      | 19.4575
      | 19.4608
      | 19.4635
      | 19.4663
      | 19.4698
      | 19.4733
      | 19.4747
      | 19.4759
      | 19.4764
      | 19.4768
      | 19.4770
      | 19.4765
      | 19.4748
      | 19.4726
      | 19.4709
      | 19.4720
      | 19.4723
      | 19.4723
      | 19.4725
      | 19.4732
      | 19.4737
      | 19.4740
      | 19.4739
      | 19.4727
      | 19.4703
      | 19.4689
      | 19.4684
      | 19.4686
      | 19.4692
      | 19.4708
      | 19.4722
      | 19.4733
      | 19.4748
      | 19.4762
      | 19.4771
      | 19.4781
      | 19.4793
      | 19.4799
      | 19.4800
      | 19.4780
      | 19.4750
      | 19.4711
      | 19.4671
      | 19.4645
      | 19.4622
      | 19.4593
      | 19.4565
      | 19.4537
      | 19.4509
      | 19.4491
      | 19.4458
      | 19.4422
      | 19.4385
      | 19.4349
      | 19.4324
      | 19.4331
      | 19.4363
      | 19.4399
      | 19.4434
      | 19.4470
      | 19.4506
      | 19.4530
      | 19.4521
      | 19.4497
      | 19.4491
      | 19.4497
      | 19.4509
      | 19.4526
      | 19.4543
      | 19.4559
      | 19.4586
      | 19.4620
      | 19.4653
      | 19.4677
      | 19.4680
      | 19.4661
      | 19.4640
      | 19.4615
      | 19.4593
      | 19.4590
      | 19.4602
      | 19.4628
      | 19.4650
      | 19.4657
      | 19.4622
      | 19.4585
      | 19.4549
      | 19.4544
      | 19.4578
      | 19.4615
      | 19.4653
      | 19.4690
      | 19.4728
      | 19.4754
      | 19.4772
      | 19.4792
      | 19.4817
      | 19.4844
      | 19.4877
      | 19.4914
      | 19.4951
      | 19.4983
      | 19.4998
      | 19.5008
      | 19.5009
      | 19.4998
      | 19.4976
      | 19.4952
      | 19.4949
      | 19.4943
      | 19.4929
      | 19.4896
      | 19.4872
      | 19.4855
      | 19.4828
      | 19.4815
      | 19.4808
      | 19.4801
      | 19.4780
      | 19.4744
      | 19.4708
      | 19.4672
      | 19.4636
      | 19.4600
      | 19.4565
      | 19.4555
      | 19.4592
      | 19.4629
      | 19.4666
      | 19.4704
      | 19.4742
      | 19.4780
      | 19.4819
      | 19.4858
      | 19.4897
      | 19.4936
      | 19.4971
      | 19.4985
      | 19.4992
      | 19.4999
      | 19.5003
      | 19.5011
      | 19.5020
      | 19.5029
      | 19.5026
      | 19.5022
      | 19.5014
      | 19.5018
      | 19.5041
      | 19.5073
      | 19.5106
      | 19.5135
      | 19.5162
      | 19.5191
      | 19.5216
      | 19.5243
      | 19.5256
      | 19.5263
      | 19.5268
      | 19.5268
      | 19.5268
      | 19.5270
      | 19.5274
      | 19.5282
      | 19.5302
      | 19.5337
      | 19.5379
      | 19.5423
      | 19.5466
      | 19.5510
      | 19.5554
      | 19.5599
      | 19.5552
      | 19.5509
      | 19.5469
      | 19.5432
      | 19.5411
      | 19.5400
      | 19.5380
      | 19.5343
      | 19.5298
      | 19.5260
      | 19.5234
      | 19.5221
      | 19.5208
      | 19.5207
      | 19.5219
      | 19.5238
      | 19.5258
      | 19.5282
      | 19.5317
      | 19.5356
      | 19.5398
      | 19.5439
      | 19.5473
      | 19.5502
      | 19.5524
      | 19.5524
      | 19.5516
      | 19.5516
      | 19.5520
      | 19.5535
      | 19.5560
      | 19.5568
      | 19.5565
      | 19.5538
      | 19.5515
      | 19.5495
      | 19.5472
      | 19.5453
      | 19.5443
      | 19.5449
      | 19.5464
      | 19.5490
      | 19.5527
      | 19.5550
      | 19.5526
      | 19.5481
      | 19.5437
      | 19.5394
      | 19.5351
      | 19.5308
      | 19.5266
      | 19.5224
      | 19.5184
      | 19.5165
      | 19.5194
      | 19.5236
      | 19.5278
      | 19.5321
      | 19.5363
      | 19.5407
      | 19.5450
      | 19.5494
      | 19.5538
      | 19.5582
      | 19.5623
      | 19.5607
      | 19.5558
      | 19.5509
      | 19.5460
      | 19.5412
      | 19.5364
      | 19.5317
      | 19.5270
      | 19.5224
      | 19.5177
      | 19.5132
      | 19.5087
      | 19.5042
      | 19.4998
      | 19.4954
      | 19.4910
      | 19.4867
      | 19.4824
      | 19.4793
      | 19.4801
      | 19.4823
      | 19.4860
      | 19.4899
      | 19.4938
      | 19.4977
      | 19.4985
      | 19.4984
      | 19.4960
      | 19.4915
      | 19.4896
      | 19.4897
      | 19.4913
      | 19.4930
      | 19.4951
      | 19.4979
      | 19.5007
      | 19.5031
      | 19.5045
      | 19.5052
      | 19.5061
      | 19.5060
      | 19.5051
      | 19.5035
      | 19.5005
      | 19.4995
      | 19.4999
      | 19.5011
      | 19.5031
      | 19.5058
      | 19.5096
      | 19.5136
      | 19.5174
      | 19.5212
      | 19.5246
      | 19.5280
      | 19.5308
      | 19.5333
      | 19.5358
      | 19.5370
      | 19.5377
      | 19.5387
      | 19.5387
      | 19.5394
      | 19.5401
      | 19.5411
      | 19.5428
      | 19.5448
      | 19.5473
      | 19.5499
      | 19.5528
      | 19.5553
      | 19.5577
      | 19.5601
      | 19.5635
      | 19.5663
      | 19.5683
      | 19.5708
      | 19.5734
      | 19.5761
      | 19.5777
      | 19.5794
      | 19.5813
      | 19.5837
      | 19.5861
      | 19.5882
      | 19.5893
      | 19.5898
      | 19.5905
      | 19.5917
      | 19.5920
      | 19.5924
      | 19.5928
      | 19.5932
      | 19.5936
      | 19.5940
      | 19.5944
      | 19.5948
      | 19.5952
      | 19.5955
      | 19.5957
      | 19.5958
      | 19.5955
      | 19.5947
      | 19.5938
      | 19.5930
      | 19.5922
      | 19.5914
      | 19.5907
      | 19.5900
      | 19.5895
      | 19.5893
      | 19.5884
      | 19.5873
      | 19.5861
      | 19.5844
      | 19.5818
      | 19.5800
      | 19.5796
      | 19.5796
      | 19.5801
      | 19.5807
      | 19.5812
      | 19.5818
      | 19.5824
      | 19.5831
      | 19.5839
      | 19.5853
      | 19.5860
      | 19.5870
      | 19.5886
      | 19.5900
      | 19.5911
      | 19.5930
      | 19.5953
      | 19.5970
      | 19.5985
      | 19.5999
      | 19.6008
      | 19.6023
      | 19.6034
      | 19.6037
      | 19.6036
      | 19.6042
      | 19.6047
      | 19.6052
      | 19.6056
      | 19.6059
      | 19.6059
      | 19.6065
      | 19.6071
      | 19.6077
      | 19.6085
      | 19.6096
      | 19.6114
      | 19.6134
      | 19.6159
      | 19.6193
      | 19.6226
      | 19.6254
      | 19.6283
      | 19.6327
      | 19.6364
      | 19.6391
      | 19.6430
      | 19.6461
      | 19.6484
      | 19.6500
      | 19.6514
      | 19.6524
      | 19.6524
      | 19.6522
      | 19.6514
      | 19.6509
      | 19.6508
      | 19.6502
      | 19.6501
      | 19.6508
      | 19.6521
      | 19.6525
      | 19.6529
      | 19.6534
      | 19.6539
      | 19.6547
      | 19.6562
      | 19.6572
      | 19.6574
      | 19.6573
      | 19.6568
      | 19.6566
      | 19.6561
      | 19.6559
      | 19.6563
      | 19.6568
      | 19.6575
      | 19.6584
      | 19.6601
      | 19.6618
      | 19.6635
      | 19.6651
      | 19.6665
      | 19.6674
      | 19.6692
      | 19.6710
      | 19.6730
      | 19.6754
      | 19.6772
      | 19.6790
      | 19.6811
      | 19.6838
      | 19.6862
      | 19.6880
      | 19.6879
      | 19.6864
      | 19.6831
      | 19.6781
      | 19.6741
      | 19.6703
      | 19.6657
      | 19.6633
      | 19.6625
      | 19.6618
      | 19.6613
      | 19.6613
      | 19.6622
      | 19.6639
      | 19.6654
      | 19.6666
      | 19.6669
      | 19.6670
      | 19.6669
      | 19.6662
      | 19.6647
      | 19.6612
      | 19.6570
      | 19.6525
      | 19.6490
      | 19.6470
      | 19.6467
      | 19.6497
      | 19.6532
      | 19.6563
      | 19.6583
      | 19.6606
      | 19.6620
      | 19.6613
      | 19.6596
      | 19.6572
      | 19.6548
      | 19.6523
      | 19.6496
      | 19.6480
      | 19.6481
      | 19.6491
      | 19.6507
      | 19.6538
      | 19.6572
      | 19.6602
      | 19.6619
      | 19.6632
      | 19.6637
      | 19.6643
      | 19.6648
      | 19.6653
      | 19.6659
      | 19.6663
      | 19.6667
      | 19.6670
      | 19.6670
      | 19.6677
      | 19.6687
      | 19.6703
      | 19.6714
      | 19.6734
      | 19.6757
      | 19.6786
      | 19.6816
      | 19.6847
      | 19.6865
      | 19.6881
      | 19.6892
      | 19.6894
      | 19.6868
      | 19.6813
      | 19.6759
      | 19.6705
      | 19.6651
      | 19.6598
      | 19.6546
      | 19.6493
      | 19.6441
      | 19.6390
      | 19.6339
      | 19.6288
      | 19.6238
      | 19.6188
      | 19.6138
      | 19.6089
      | 19.6041
      | 19.5993
      | 19.5945
      | 19.5898
      | 19.5851
      | 19.5805
      | 19.5759
      | 19.5714
      | 19.5669
      | 19.5624
      | 19.5580
      | 19.5536
      | 19.5493
      | 19.5450
      | 19.5407
      | 19.5365
      | 19.5323
      | 19.5282
      | 19.5241
      | 19.5200
      | 19.5160
      | 19.5120
      | 19.5080
      | 19.5040
      | 19.5000
      | 19.4961
      | 19.4922
      | 19.4883
      | 19.4845
      | 19.4806
      | 19.4768
      | 19.4730
      | 19.4692
      | 19.4654
      | 19.4617
      | 19.4580
      | 19.4543
      | 19.4506
      | 19.4470
      | 19.4456
      | 19.4491
      | 19.4528
      | 19.4564
      | 19.4601
      | 19.4638
      | 19.4675
      | 19.4713
      | 19.4751
      | 19.4789
      | 19.4827
      | 19.4866
      | 19.4905
      | 19.4945
      | 19.4985
      | 19.5025
      | 19.5065
      | 19.5105
      | 19.5145
      | 19.5173
      | 19.5198
      | 19.5227
      | 19.5251
      | 19.5275
      | 19.5300
      | 19.5325
      | 19.5352
      | 19.5382
      | 19.5421
      | 19.5459
      | 19.5491
      | 19.5522
      | 19.5563
      | 19.5604
      | 19.5620
      | 19.5633
      | 19.5639
      | 19.5644
      | 19.5645
      | 19.5640
      | 19.5621
      | 19.5596
      | 19.5576
      | 19.5589
      | 19.5593
      | 19.5592
      | 19.5595
      | 19.5602
      | 19.5608
      | 19.5612
      | 19.5610
      | 19.5596
      | 19.5569
      | 19.5553
      | 19.5548
      | 19.5550
      | 19.5557
      | 19.5574
      | 19.5590
      | 19.5602
      | 19.5620
      | 19.5636
      | 19.5645
      | 19.5656
      | 19.5670
      | 19.5676
      | 19.5677
      | 19.5655
      | 19.5621
      | 19.5577
      | 19.5532
      | 19.5502
      | 19.5476
      | 19.5444
      | 19.5412
      | 19.5381
      | 19.5348
      | 19.5328
      | 19.5291
      | 19.5250
      | 19.5208
      | 19.5167
      | 19.5138
      | 19.5147
      | 19.5184
      | 19.5226
      | 19.5268
      | 19.5310
      | 19.5353
      | 19.5380
      | 19.5369
      | 19.5343
      | 19.5335
      | 19.5342
      | 19.5356
      | 19.5374
      | 19.5393
      | 19.5412
      | 19.5443
      | 19.5482
      | 19.5519
      | 19.5548
      | 19.5550
      | 19.5528
      | 19.5505
      | 19.5477
      | 19.5452
      | 19.5448
      | 19.5461
      | 19.5491
      | 19.5516
      | 19.5523
      | 19.5484
      | 19.5443
      | 19.5402
      | 19.5396
      | 19.5435
      | 19.5479
      | 19.5523
      | 19.5567
      | 19.5612
      | 19.5641
      | 19.5662
      | 19.5684
      | 19.5713
      | 19.5744
      | 19.5781
      | 19.5824
      | 19.5868
      | 19.5905
      | 19.5922
      | 19.5933
      | 19.5933
      | 19.5921
      | 19.5896
      | 19.5869
      | 19.5866
      | 19.5858
      | 19.5842
      | 19.5805
      | 19.5778
      | 19.5759
      | 19.5728
      | 19.5713
      | 19.5704
      | 19.5696
      | 19.5673
      | 19.5632
      | 19.5591
      | 19.5550
      | 19.5510
      | 19.5469
      | 19.5429
      | 19.5418
      | 19.5461
      | 19.5505
      | 19.5549
      | 19.5594
      | 19.5639
      | 19.5684
      | 19.5729
      | 19.5775
      | 19.5822
      | 19.5868
      | 19.5908
      | 19.5924
      | 19.5932
      | 19.5939
      | 19.5944
      | 19.5954
      | 19.5964
      | 19.5973
      | 19.5971
      | 19.5966
      | 19.5956
      | 19.5961
      | 19.5987
      | 19.6023
      | 19.6062
      | 19.6095
      | 19.6125
      | 19.6159
      | 19.6188
      | 19.6218
      | 19.6234
      | 19.6241
      | 19.6247
      | 19.6246
      | 19.6247
      | 19.6249
      | 19.6253
      | 19.6262
      | 19.6285
      | 19.6325
      | 19.6375
      | 19.6426
      | 19.6477
      | 19.6529
      | 19.6581
      | 19.6633
      | 19.6580
      | 19.6533
      | 19.6488
      | 19.6446
      | 19.6424
      | 19.6411
      | 19.6389
      | 19.6348
      | 19.6298
      | 19.6255
      | 19.6226
      | 19.6211
      | 19.6197
      | 19.6196
      | 19.6210
      | 19.6231
      | 19.6254
      | 19.6282
      | 19.6322
      | 19.6367
      | 19.6417
      | 19.6464
      | 19.6504
      | 19.6537
      | 19.6562
      | 19.6562
      | 19.6554
      | 19.6555
      | 19.6560
      | 19.6577
      | 19.6606
      | 19.6615
      | 19.6612
      | 19.6583
      | 19.6557
      | 19.6535
      | 19.6510
      | 19.6490
      | 19.6479
      | 19.6486
      | 19.6503
      | 19.6533
      | 19.6576
      | 19.6602
      | 19.6577
      | 19.6528
      | 19.6480
      | 19.6432
      | 19.6384
      | 19.6338
      | 19.6291
      | 19.6246
      | 19.6202
      | 19.6181
      | 19.6215
      | 19.6265
      | 19.6315
      | 19.6365
      | 19.6416
      | 19.6467
      | 19.6519
      | 19.6570
      | 19.6623
      | 19.6675
      | 19.6723
      | 19.6706
      | 19.6652
      | 19.6599
      | 19.6546
      | 19.6494
      | 19.6442
      | 19.6391
      | 19.6340
      | 19.6289
      | 19.6239
      | 19.6189
      | 19.6140
      | 19.6091
      | 19.6043
      | 19.5995
      | 19.5948
      | 19.5901
      | 19.5855
      | 19.5821
      | 19.5831
      | 19.5857
      | 19.5902
      | 19.5949
      | 19.5996
      | 19.6043
      | 19.6053
      | 19.6053
      | 19.6027
      | 19.5979
      | 19.5960
      | 19.5961
      | 19.5981
      | 19.6002
      | 19.6027
      | 19.6061
      | 19.6094
      | 19.6123
      | 19.6139
      | 19.6149
      | 19.6161
      | 19.6162
      | 19.6153
      | 19.6137
      | 19.6105
      | 19.6095
      | 19.6101
      | 19.6117
      | 19.6141
      | 19.6173
      | 19.6220
      | 19.6267
      | 19.6313
      | 19.6358
      | 19.6399
      | 19.6439
      | 19.6473
      | 19.6503
      | 19.6533
      | 19.6549
      | 19.6559
      | 19.6572
      | 19.6575
      | 19.6584
      | 19.6594
      | 19.6608
      | 19.6629
      | 19.6653
      | 19.6684
      | 19.6716
      | 19.6751
      | 19.6781
      | 19.6810
      | 19.6839
      | 19.6881
      | 19.6915
      | 19.6939
      | 19.6970
      | 19.7001
      | 19.7035
      | 19.7055
      | 19.7077
      | 19.7101
      | 19.7131
      | 19.7160
      | 19.7186
      | 19.7202
      | 19.7210
      | 19.7220
      | 19.7236
      | 19.7243
      | 19.7251
      | 19.7258
      | 19.7266
      | 19.7273
      | 19.7281
      | 19.7288
      | 19.7295
      | 19.7303
      | 19.7309
      | 19.7315
      | 19.7319
      | 19.7320
      | 19.7314
      | 19.7308
      | 19.7302
      | 19.7296
      | 19.7291
      | 19.7287
      | 19.7283
      | 19.7281
      | 19.7282
      | 19.7276
      | 19.7269
      | 19.7259
      | 19.7244
      | 19.7219
      | 19.7203
      | 19.7203
      | 19.7207
      | 19.7217
      | 19.7228
      | 19.7238
      | 19.7249
      | 19.7260
      | 19.7272
      | 19.7286
      | 19.7305
      | 19.7317
      | 19.7333
      | 19.7355
      | 19.7376
      | 19.7393
      | 19.7419
      | 19.7449
      | 19.7472
      | 19.7495
      | 19.7515
      | 19.7530
      | 19.7552
      | 19.7569
      | 19.7577
      | 19.7582
      | 19.7593
      | 19.7605
      | 19.7615
      | 19.7625
      | 19.7634
      | 19.7640
      | 19.7652
      | 19.7665
      | 19.7678
      | 19.7692
      | 19.7710
      | 19.7736
      | 19.7765
      | 19.7798
      | 19.7842
      | 19.7884
      | 19.7922
      | 19.7961
      | 19.8016
      | 19.8064
      | 19.8099
      | 19.8149
      | 19.8191
      | 19.8223
      | 19.8247
      | 19.8269
      | 19.8287
      | 19.8295
      | 19.8299
      | 19.8298
      | 19.8300
      | 19.8306
      | 19.8308
      | 19.8314
      | 19.8330
      | 19.8351
      | 19.8363
      | 19.8375
      | 19.8389
      | 19.8403
      | 19.8420
      | 19.8444
      | 19.8463
      | 19.8473
      | 19.8481
      | 19.8484
      | 19.8491
      | 19.8494
      | 19.8500
      | 19.8514
      | 19.8529
      | 19.8544
      | 19.8564
      | 19.8591
      | 19.8619
      | 19.8647
      | 19.8673
      | 19.8698
      | 19.8718
      | 19.8747
      | 19.8776
      | 19.8808
      | 19.8844
      | 19.8873
      | 19.8904
      | 19.8936
      | 19.8976
      | 19.9013
      | 19.9043
      | 19.9053
      | 19.9046
      | 19.9022
      | 19.8980
      | 19.8948
      | 19.8918
      | 19.8880
      | 19.8866
      | 19.8868
      | 19.8872
      | 19.8879
      | 19.8891
      | 19.8912
      | 19.8942
      | 19.8971
      | 19.8996
      | 19.9011
      | 19.9025
      | 19.9036
      | 19.9042
      | 19.9038
      | 19.9014
      | 19.8982
      | 19.8947
      | 19.8922
      | 19.8915
      | 19.8924
      | 19.8971
      | 19.9022
      | 19.9070
      | 19.9105
      | 19.9144
      | 19.9173
      | 19.9181
      | 19.9177
      | 19.9166
      | 19.9155
      | 19.9143
      | 19.9129
      | 19.9127
      | 19.9144
      | 19.9170
      | 19.9203
      | 19.9252
      | 19.9305
      | 19.9354
      | 19.9387
      | 19.9418
      | 19.9440
      | 19.9463
      | 19.9485
      | 19.9508
      | 19.9530
      | 19.9553
      | 19.9574
      | 19.9595
      | 19.9612
      | 19.9638
      | 19.9667
      | 19.9702
      | 19.9732
      | 19.9772
      | 19.9816
      | 19.9866
      | 19.9917
      | 19.9970
      | 20.0008
      | 20.0045
      | 20.0077
      | 20.0099
      | 20.0092
      | 20.0055
      | 20.0018
      | 19.9983
      | 19.9948
      | 19.9913
      | 19.9879
      | 19.9846
      | 19.9813
      | 19.9782
      | 19.9750
      | 19.9720
      | 19.9690
      | 19.9661
      | 19.9633
      | 19.9605
      | 19.9578
      | 19.9552
      | 19.9526
      | 19.9502
      | 19.9478
      | 19.9455
      | 19.9432
      | 19.9411
      | 19.9391
      | 19.9371
      | 19.9352
      | 19.9334
      | 19.9317
      | 19.9301
      | 19.9285
      | 19.9270
      | 19.9256
      | 19.9242
      | 19.9229
      | 19.9216
      | 19.9203
      | 19.9191
      | 19.9179
      | 19.9168
      | 19.9158
      | 19.9147
      | 19.9138
      | 19.9129
      | 19.9120
      | 19.9112
      | 19.9104
      | 19.9097
      | 19.9091
      | 19.9085
      | 19.9079
      | 19.9074
      | 19.9070
      | 19.9066
      | 19.9063
      | 19.9083
      | 19.9156
      | 19.9229
      | 19.9303
      | 19.9378
      | 19.9453
      | 19.9529
      | 19.9606
      | 19.9683
      | 19.9761
      | 19.9840
      | 19.9919
      | 19.9998
      | 20.0079
      | 20.0160
      | 20.0241
      | 20.0324
      | 20.0406
      | 20.0487
      | 20.0557
      | 20.0624
      | 20.0695
      | 20.0761
      | 20.0828
      | 20.0896
      | 20.0965
      | 20.1035
      | 20.1110
      | 20.1195
      | 20.1278
      | 20.1355
      | 20.1432
      | 20.1520
      | 20.1608
      | 20.1670
      | 20.1730
      | 20.1783
      | 20.1835
      | 20.1884
      | 20.1927
      | 20.1956
      | 20.1981
      | 20.2010
      | 20.2072
      | 20.2127
      | 20.2177
      | 20.2231
      | 20.2289
      | 20.2348
      | 20.2404
      | 20.2455
      | 20.2495
      | 20.2522
      | 20.2561
      | 20.2612
      | 20.2675
      | 20.2743
      | 20.2821
      | 20.2899
      | 20.2974
      | 20.3054
      | 20.3133
      | 20.3208
      | 20.3284
      | 20.3363
      | 20.3435
      | 20.3504
      | 20.3550
      | 20.3586
      | 20.3612
      | 20.3639
      | 20.3680
      | 20.3725
      | 20.3765
      | 20.3806
      | 20.3847
      | 20.3888
      | 20.3941
      | 20.3979
      | 20.4012
      | 20.4046
      | 20.4081
      | 20.4128
      | 20.4212
      | 20.4323
      | 20.4438
      | 20.4555
      | 20.4673
      | 20.4791
      | 20.4897
      | 20.4968
      | 20.5024
      | 20.5100
      | 20.5189
      | 20.5286
      | 20.5387
      | 20.5490
      | 20.5593
      | 20.5708
      | 20.5831
      | 20.5953
      | 20.6068
      | 20.6160
      | 20.6231
      | 20.6301
      | 20.6367
      | 20.6437
      | 20.6527
      | 20.6633
      | 20.6755
      | 20.6874
      | 20.6978
      | 20.7038
      | 20.7096
      | 20.7153
      | 20.7243
      | 20.7378
      | 20.7518
      | 20.7659
      | 20.7802
      | 20.7945
      | 20.8073
      | 20.8195
      | 20.8319
      | 20.8449
      | 20.8583
      | 20.8724
      | 20.8871
      | 20.9019
      | 20.9162
      | 20.9287
      | 20.9407
      | 20.9518
      | 20.9619
      | 20.9709
      | 20.9798
      | 20.9910
      | 21.0019
      | 21.0120
      | 21.0204
      | 21.0299
      | 21.0401
      | 21.0494
      | 21.0602
      | 21.0717
      | 21.0834
      | 21.0938
      | 21.1028
      | 21.1118
      | 21.1210
      | 21.1303
      | 21.1397
      | 21.1493
      | 21.1616
      | 21.1790
      | 21.1966
      | 21.2143
      | 21.2321
      | 21.2501
      | 21.2683
      | 21.2865
      | 21.3050
      | 21.3235
      | 21.3422
      | 21.3604
      | 21.3765
      | 21.3921
      | 21.4077
      | 21.4232
      | 21.4393
      | 21.4555
      | 21.4719
      | 21.4873
      | 21.5026
      | 21.5177
      | 21.5341
      | 21.5526
      | 21.5721
      | 21.5919
      | 21.6114
      | 21.6307
      | 21.6505
      | 21.6700
      | 21.6898
      | 21.7084
      | 21.7266
      | 21.7446
      | 21.7623
      | 21.7802
      | 21.7984
      | 21.8168
      | 21.8357
      | 21.8554
      | 21.8755
      | 21.8951
      | 21.9147
      | 21.9330
      | 21.9504
      | 21.9682
      | 21.9862
      | 22.0048
      | 22.0232
      | 22.0418
      | 22.0608
      | 22.0803
      | 22.0998
      | 22.1208
      | 22.1429
      | 22.1663
      | 22.1904
      | 22.2150
      | 22.2387
      | 22.2623
      | 22.2859
      | 22.3088
      | 22.3323
      | 22.3556
      | 22.3793
      | 22.4037
      | 22.4285
      | 22.4539
      | 22.4793
      | 22.5043
      | 22.5285
      | 22.5504
      | 22.5721
      | 22.5941
      | 22.6163
      | 22.6388
      | 22.6616
      | 22.6846
      | 22.7080
      | 22.7315
      | 22.7554
      | 22.7794
      | 22.8038
      | 22.8284
      | 22.8533
      | 22.8785
      | 22.9039
      | 22.9296
      | 22.9555
      | 22.9818
      | 23.0083
      | 23.0351
      | 23.0621
      | 23.0895
      | 23.1170
      | 23.1449
      | 23.1730
      | 23.2014
      | 23.2301
      | 23.2591
      | 23.2883
      | 23.3179
      | 23.3477
      | 23.3779
      | 23.4084
      | 23.4392
      | 23.4705
      | 23.5021
      | 23.5341
      | 23.5665
      | 23.5993
      | 23.6325
      | 23.6661
      | 23.7001
      | 23.7344
      | 23.7692
      | 23.8043
      | 23.8399
      | 23.8758
      | 23.9121
      | 23.9489
      | 23.9860
      | 24.0235
      | 24.0615
      | 24.0998
      | 24.1385
      | 24.1777
      | 24.2172
      | 24.2571
      | 24.2975
      | 24.3383
      | 24.3794
      | 24.4210
      | 24.4630
      | 24.5054
      | 24.5483
      | 24.5915
      | 24.6352
      | 24.6793
      | 24.7238
      | 24.7688
      | 24.8142
      | 24.8600
      | 24.9063
      | 24.9529
      | 25.0000
      | ]
  SOC-Vol : Lookup_n-D  NumberOfTableDimensions=1  BreakpointsForDimension1=battery_SOC_SOC  Table=battery_SOC_voltage  ExtrapMethod=Clip  RemoveProtectionInput=on  UseLastTableValue=on  InternalRulePriority=Speed  RndMeth=Simplest
  SOC_t-1 : UnitDelay  SampleTime=-1  HasFrameUpgradeWarning=on
  Saturation1 : Saturate  UpperLimit=100  LowerLimit=0
  Signal Specification4 : SignalSpecification  Unit=m/s
  Signal Specification5 : SignalSpecification  Unit=km/hr
  Signal Specification8 : SignalSpecification  Unit=rpm
  Signal Specification9 : SignalSpecification  Unit=rad/s
  Speed Different : Sum  Inputs=+-
  Square1 : Math  Operator=square
  Step : Step  Time=10  SampleTime=0
  Sum : Sum  Inputs=|+-
  Switch1 : Switch  Criteria=u2 ~= 0  SaturateOnIntegerOverflow=off  InputSameDT=off
  Unit Conversion2 : UnitConversion
  Unit Conversion4 : UnitConversion
  Vol-R : Lookup_n-D  NumberOfTableDimensions=1  BreakpointsForDimension1=battery_SOC_SOC  Table=battery_SOC_resistance  RemoveProtectionInput=on  InternalRulePriority=Speed  RndMeth=Simplest
  Vol_pack : Gain  Gain=100
  Zero-Order Hold : ZeroOrderHold  SampleTime=0.1
  Zero-Order Hold1 : ZeroOrderHold  SampleTime=0.1
  Accel[m/s2] : Outport
  Speed[m/s] : Outport  Port=2
  Position[m] : Outport  Port=3
  Battery_SOC[%] : Outport  Port=4
  Temperature_cell : Outport  Port=5
  Voltage_cell : Outport  Port=6
  Current_cell : Outport  Port=7
  wires:
  Discrete-Time Integrator1/1 -> Position[m]/1, Sum/1
  Unit Conversion2/1 -> Signal Specification5/1
  From Workspace9/1 -> Divide15/2
  Divide15/1 -> [Accel_ms2], Accel[m/s2]/1, Discrete-Time Integrator/1  "Veh_acceleartion"
  pos_follow/1 -> Sum/2
  Discrete-Time Integrator/1 -> Signal Specification4/1
  Signal Specification4/1 -> [Speed_ms], Speed[m/s]/1, Discrete-Time Integrator1/1, Unit Conversion2/1
  PID Controller/1 -> Brake[%]1/1, Accel[%]1/1  "Acceleration"
  Signal Specification5/1 -> [Speed]
  Speed Different/1 -> PID Controller/1  "Speed Different"
  Target speed/1 -> Speed Different/1
  [Speed] -> Speed Different/2
  Gain17/1 -> Current_cell/1, " Normalization"/3(Current), Coulomb Counting/1(Motor_Current_cell)  "Motor_Current_cell"
  [Electric_Power] -> Divide12/1
  " Normalization"/2(Voltage_n) -> Mux2/2
  LSTM/1(SOC) -> Zero-Order Hold1/1  "predictedSOC"
  Vol_pack/1 -> Divide12/2
  Vol-R/1 -> Divide11/2
  SOC_t-1/1 -> SOC-Vol/1, SOC-Temp/1
